simulink model "MATLAB_TEST"  (R2019b)
settings: Solver=FixedStepDiscrete  StartTime=0  StopTime=50  FixedStep=0.0025  RelTol=1e-3
undefined symbols (not defined in the file): BCM_COM_PROC_P20, BCM_COM_PROC_P20_SFW_R2018b, BCM_COM_PROC_P2_5, BCM_COM_PROC_P2_5_SFW_R2018b, BCM_COM_PROC_P5, BCM_COM_PROC_P5_SFW_R2018b, BCMA_ACCU_PT_Conf_Flt, BCMA_ACCU_PT_Unconf_Flt, BCMA_Antiskid_Off_Sanction, BCMA_Avionics_Conf_Flt, BCMA_BCM_CCDL_Conf_Flt, BCMA_BCM_CCDL_Unconf_Flt, BCMA_BCM_DBCU_INHIBITION_Conf_Flt, BCMA_BCM_DBCU_INHIBITION_Unconf_Flt, BCMA_BCP_ALT_Disp_Sw_Conf_Flt, BCMA_BCP_ALT_Disp_Sw_Unconf_Flt, BCMA_BCP_ALT_SW_ON_CMD_Conf_Flt, BCMA_BCP_ALT_SW_ON_CMD_Unconf_Flt, BCMA_BCP_PARK_OFF_SW_CMD_Conf_Flt, BCMA_BCP_PARK_OFF_SW_CMD_Unconf_Flt, BCMA_CF_BSELV_JCL, BCMA_CF_BSELV_JOP, BCMA_CF_BSELV_OC, BCMA_CF_BSELV_SC, BCMA_CF_LH_SV_JCL, BCMA_CF_LH_SV_JOP, BCMA_CF_LH_SV_OC, BCMA_CF_LH_SV_SC, BCMA_CF_PARK_BRK, BCMA_CF_RESIDUAL_PRESS, BCMA_CF_RH_SV_JCL, BCMA_CF_RH_SV_JOP, BCMA_CF_RH_SV_OC, BCMA_CF_RH_SV_SC, BCMA_CF_SELV_JCL, BCMA_CF_SELV_JOP, BCMA_CF_SELV_OC, BCMA_CF_SELV_SC, BCMA_CF_SV_DRIFT, BCMA_DBCU_ALT_MODE_Conf_Flt, BCMA_DBCU_ALT_MODE_Unconf_Flt, BCMA_DBCU_BRK_ORDER_FAIL_Conf_Flt, BCMA_DBCU_BRK_ORDER_FAIL_Unconf_Flt, BCMA_DBCU_Conf_Flt, BCMA_DBCU_DISPATCH_SW_ON_Conf_Flt, BCMA_DBCU_DISPATCH_SW_ON_Unconf_Flt, BCMA_DBCU_FAILED_Conf_Flt, BCMA_DBCU_FAILED_Unconf_Flt, BCMA_DFCS1_Capsule_Validity, BCMA_DFCS1_Label202_Corrupted, BCMA_DFCS1_Label202_Not_Refreshed, BCMA_DFCS1_Label204_Corrupted, BCMA_DFCS1_Label204_Not_Refreshed, BCMA_DFCS1_Label205_Corrupted, BCMA_DFCS1_Label205_Not_Refreshed, BCMA_DFCS1_Label206_Corrupted, BCMA_DFCS1_Label206_Not_Refreshed, BCMA_DFCS1_Label207_Corrupted, BCMA_DFCS1_Label207_Not_Refreshed, BCMA_DFCS3_Capsule_Validity ... (+762)
libraries: simulink x73, lib_MBD_Control x5
(part 5 of 16)

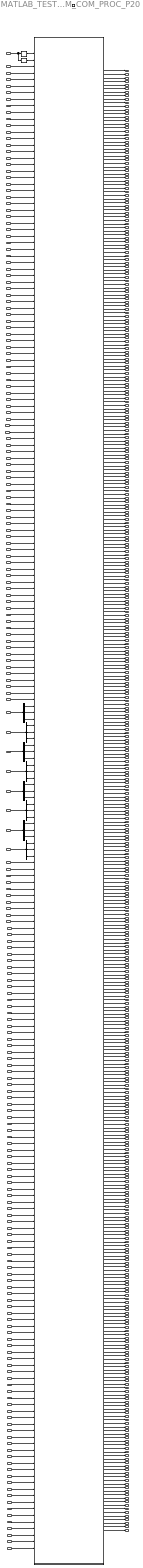
== system MATLAB_TEST/AVIONICS/Brake_Control_Module_Side_A/BCSA Controller CP/BCM_COM_PROC_P20 ==
  V_BCM_COM_Tachometers_Conf_Flt : Inport
  V_BCM_COM_DFCS_A_Gnd_Spd_Acq : Inport  Port=2
  V_BCM_COM_DFCS_B_Gnd_Spd_Acq : Inport  Port=3
  V_BCM_COM_DFCS_A_Gnd_Spd_Val : Inport  Port=4
  V_BCM_COM_DFCS_B_Gnd_Spd_Val : Inport  Port=5
  V_BCM_COM_DFCS_A_Long_Accel_Acq : Inport  Port=6
  V_BCM_COM_DFCS_B_Long_Accel_Acq : Inport  Port=7
  V_BCM_COM_DFCS_A_AC_Long_Accel_Val : Inport  Port=8
  V_BCM_COM_DFCS_B_AC_Long_Accel_Val : Inport  Port=9
  V_BCM_COM_DFCS_A_Pitch_Ang_Acq : Inport  Port=10
  V_BCM_COM_DFCS_B_Pitch_Ang_Acq : Inport  Port=11
  V_BCM_COM_DFCS_A_AC_Pitch_Angle_Val : Inport  Port=12
  V_BCM_COM_DFCS_B_AC_Pitch_Angle_Val : Inport  Port=13
  V_BCM_COM_DFCS_A_WOWs_Val_Acq : Inport  Port=14
  V_BCM_COM_DFCS_B_WOWs_Val_Acq : Inport  Port=15
  V_BCM_COM_DFCS_A_WOWs_Val_Val : Inport  Port=16
  V_BCM_COM_DFCS_B_WOWs_Val_Val : Inport  Port=17
  V_BCM_COM_DFCS_A_LMLG_WOWs_Val : Inport  Port=18
  V_BCM_COM_DFCS_B_LMLG_WOWs_Val : Inport  Port=19
  V_BCM_COM_DFCS_A_LMLG_WOWs_Acq : Inport  Port=20
  V_BCM_COM_DFCS_B_LMLG_WOWs_Acq : Inport  Port=21
  V_BCM_COM_DFCS_A_RMLG_WOWs_Val : Inport  Port=22
  V_BCM_COM_DFCS_B_RMLG_WOWs_Val : Inport  Port=23
  V_BCM_COM_DFCS_A_RMLG_WOWs_Acq : Inport  Port=24
  V_BCM_COM_DFCS_B_RMLG_WOWs_Acq : Inport  Port=25
  V_BCM_COM_DFCS_A_NLG_WOWs_Val : Inport  Port=26
  V_BCM_COM_DFCS_B_NLG_WOWs_Val : Inport  Port=27
  V_BCM_COM_DFCS_A_NLG_WOWs_Acq : Inport  Port=28
  V_BCM_COM_DFCS_B_NLG_WOWs_Acq : Inport  Port=29
  V_BCM_COM_RH_Decel_Law_Brkg_Press_Cmd : Inport  Port=30
  V_BCM_COM_LH_Decel_Law_Brkg_Press_Cmd : Inport  Port=31
  V_BCM_COM_Hyd_A_Press_Acq : Inport  Port=32
  V_BCM_COM_Hyd_B_Press_Acq : Inport  Port=33
  V_BCM_COM_DFCS_A_LH_Braking_Cmd_Val : Inport  Port=34
  V_BCM_COM_DFCS_A_RH_Braking_Cmd_Val : Inport  Port=35
  V_BCM_COM_DFCS_B_LH_Braking_Cmd_Val : Inport  Port=36
  V_BCM_COM_DFCS_B_RH_Braking_Cmd_Val : Inport  Port=37
  V_BCM_COM_DFCS_A_DFCS_LH_Braking_Cmd_Acq : Inport  Port=38
  V_BCM_COM_DFCS_A_DFCS_RH_Braking_Cmd_Acq : Inport  Port=39
  V_BCM_COM_DFCS_B_DFCS_LH_Braking_Cmd_Acq : Inport  Port=40
  V_BCM_COM_DFCS_B_DFCS_RH_Braking_Cmd_Acq : Inport  Port=41
  V_BCM_COM_DFCS_A_Decel_Law_Inhib_Val : Inport  Port=42
  V_BCM_COM_DFCS_A_Decel_Law_Inhib_Acq : Inport  Port=43
  V_BCM_COM_DFCS_B_Decel_Law_Inhib_Val : Inport  Port=44
  V_BCM_COM_DFCS_B_Decel_Law_Inhib_Acq : Inport  Port=45
  V_BCM_COM_DFCS_A_TLA_Above_Idle_Val : Inport  Port=46
  V_BCM_COM_DFCS_B_TLA_Above_Idle_Val : Inport  Port=47
  V_BCM_COM_DFCS_A_TLA_Above_Idle_Acq : Inport  Port=48
  V_BCM_COM_DFCS_B_TLA_Above_Idle_Acq : Inport  Port=49
  V_BCM_COM_LG_Lever_Up_Acq : Inport  Port=50
  V_BCM_COM_LG_Lever_Up_Unconf_Flt : Inport  Port=51
  V_BCM_COM_LG_Lever_Up_Conf_Flt : Inport  Port=52
  V_BCM_COM_LMLG_Downlock_Acq : Inport  Port=53
  V_BCM_COM_RMLG_Downlock_Acq : Inport  Port=54
  V_BCM_COM_LMLG_Dnlk_Unconf_Flt : Inport  Port=55
  V_BCM_COM_LMLG_Dnlk_Conf_Flt : Inport  Port=56
  V_BCM_COM_RMLG_Dnlk_Unconf_Flt : Inport  Port=57
  V_BCM_COM_RMLG_Dnlk_Conf_Flt : Inport  Port=58
  V_BCM_COM_Engine_Running_Acq : Inport  Port=59
  V_BCM_COM_PBSELV_ON_POS_Acq : Inport  Port=60
  V_BCM_COM_PBSELV_ON_POS_Unconf_Flt : Inport  Port=61
  V_BCM_COM_PBSELV_ON_POS_Conf_Flt : Inport  Port=62
  V_BCM_COM_Maint_Itv_Function_Req : Inport  Port=63
  V_BCM_COM_BCM_Config : Inport  Port=64
  V_BCM_COM_BCM_Off_Sanction : Inport  Port=65
  V_BCM_COM_BCM_Validity_By_SP : Inport  Port=66
  V_BCM_COM_BCP_BCM_Alt_Sw_On_Cmd_Acq : Inport  Port=67
  V_BCM_COM_BCP_BCM_Alt_Sw_On_Cmd_Conf_Flt : Inport  Port=68
  V_BCM_COM_BCP_BCM_Alt_Sw_On_Cmd_Unconf_Flt : Inport  Port=69
  V_BCM_COM_MP_BCMA_Alt_Disp_Sw_Conf_Flt : Inport  Port=70
  V_BCM_COM_MP_BCMA_Alt_Disp_Sw_Unconf_Flt : Inport  Port=71
  V_BCM_COM_MP_BCMA_Alt_Disp_Sw_Acq : Inport  Port=72
  V_BCM_COM_Antiskid_Off_Sanction : Inport  Port=73
  V_BCM_COM_Norm_Brkg_Off_Sanc : Inport  Port=74
  V_BCM_COM_CF_LH_ALT_BRK_LOSS : Inport  Port=75
  V_BCM_COM_CF_DBCU_FAILED : Inport  Port=76
  V_BCM_COM_CF_RH_ALT_BRK_LOSS : Inport  Port=77
  V_BCM_COM_SV_PT_Filt : Inport  Port=78
  V_BCM_COM_Whl_AS_Inhib_Cond_W12 : Inport  Port=79
  V_BCM_COM_Whl_AS_Inhib_Cond_W34 : Inport  Port=80
  V_BCM_COM_Whl_LP_AS_Curr_Order : Inport  Port=81
  V_BCM_COM_SV_PT_Cons : Inport  Port=82
  V_BCM_COM_Wheel_Filtered_Speed_W12 : Inport  Port=83
  V_BCM_COM_Wheel_Filtered_Speed_W34 : Inport  Port=84
  V_BCM_COM_Wheel_Speed_Error_W12 : Inport  Port=85
  V_BCM_COM_Wheel_Speed_Error_W34 : Inport  Port=86
  V_BCM_COM_Whl_LP_AS_Curr_Order_W12 : Inport  Port=87
  V_BCM_COM_Whl_LP_AS_Curr_Order_W34 : Inport  Port=88
  V_BCM_COM_SV_Current : Inport  Port=89
  V_BCM_COM_SV_PT_Cons_Val : Inport  Port=90
  V_BCM_COM_Opt_Adhesion_In_Acq_W12 : Inport  Port=91
  V_BCM_COM_Opt_Adhesion_In_Acq_W34 : Inport  Port=92
  V_BCM_COM_Adhesion_In_Acq_W12 : Inport  Port=93
  V_BCM_COM_Adhesion_In_Acq_W34 : Inport  Port=94
  V_BCM_COM_Target_Speed_In_Acq_W12 : Inport  Port=95
  V_BCM_COM_Target_Speed_In_Acq_W34 : Inport  Port=96
  V_BCM_COM_Big_Gamma_Trig_In_Acq_W12 : Inport  Port=97
  V_BCM_COM_Big_Gamma_Trig_In_Acq_W34 : Inport  Port=98
  V_BCM_COM_Small_Slip_Trig_In_Acq_W12 : Inport  Port=99
  V_BCM_COM_Small_Slip_Trig_In_Acq_W34 : Inport  Port=100
  V_BCM_COM_Big_Slip_Trig_In_Acq_W12 : Inport  Port=101
  V_BCM_COM_Big_Slip_Trig_In_Acq_W34 : Inport  Port=102
  V_BCM_COM_BCM_CCDL_Conf_Flt : Inport  Port=103
  V_BCM_COM_BCM_CCDL_Unconf_Flt : Inport  Port=104
  V_BCM_COM_Big_Slip_WD_Trig_In_Acq_W12 : Inport  Port=105
  V_BCM_COM_Big_Slip_WD_Trig_In_Acq_W34 : Inport  Port=106
  V_BCM_COM_BCM_DBCU_INHIBITION_Conf_Flt : Inport  Port=107
  V_BCM_COM_BCM_DBCU_INHIBITION_Unconf_Flt : Inport  Port=108
  V_BCM_COM_BCM_DBCU_INHIBITION_Acq : Inport  Port=109
  V_BCM_COM_Engine_1_Running_Acq_Val : Inport  Port=110
  V_BCM_COM_Engine_2_Running_Acq_Val : Inport  Port=111
  V_BCM_COM_Hyd_A_Press_Acq_Val : Inport  Port=112
  V_BCM_COM_Hyd_B_Press_Acq_Val : Inport  Port=113
  V_BCM_COM_DFCS_A_DBCU_ALT_Mode_1_Acq_Val : Inport  Port=114
  V_BCM_COM_DFCS_A_DBCU_ALT_Mode_2_Acq_Val : Inport  Port=115
  V_BCM_COM_DFCS_B_DBCU_ALT_Mode_1_Acq_Val : Inport  Port=116
  V_BCM_COM_DFCS_B_DBCU_ALT_Mode_2_Acq_Val : Inport  Port=117
  V_BCM_COM_UTC_Time_Hours_Acq : Inport  Port=118
  V_BCM_COM_UTC_Time_Hours_Conf_Flt : Inport  Port=119
  V_BCM_COM_UTC_Time_Hours_Unconf_Flt : Inport  Port=120
  V_BCM_COM_UTC_Time_Minutes_Acq : Inport  Port=121
  V_BCM_COM_UTC_Time_Minutes_Conf_Flt : Inport  Port=122
  V_BCM_COM_UTC_Time_Minutes_Unconf_Flt : Inport  Port=123
  V_BCM_COM_UTC_Time_Seconds_Acq : Inport  Port=124
  V_BCM_COM_UTC_Time_Seconds_Conf_Flt : Inport  Port=125
  V_BCM_COM_UTC_Time_Seconds_Unconf_Flt : Inport  Port=126
  V_BCM_COM_DBCU_BRK_ORDER_FAIL_Acq : Inport  Port=127
  V_BCM_COM_DBCU_DISPATCH_SW_ON_Acq : Inport  Port=128
  V_BCM_COM_LH_DBCU_BRK_CMD_FDBK_Acq : Inport  Port=129
  V_BCM_COM_RH_DBCU_BRK_CMD_FDBK_Acq : Inport  Port=130
  V_BCM_COM_DBCU_FAILED_Acq : Inport  Port=131
  V_BCM_COM_DBCU_ALT_MODE_Acq : Inport  Port=132
  V_BCM_COM_DBCU_BRK_ORDER_FAIL_Conf_Flt : Inport  Port=133
  V_BCM_COM_DBCU_BRK_ORDER_FAIL_Unconf_Flt : Inport  Port=134
  V_BCM_COM_DBCU_DISPATCH_SW_ON_Conf_Flt : Inport  Port=135
  V_BCM_COM_DBCU_DISPATCH_SW_ON_Unconf_Flt : Inport  Port=136
  V_BCM_COM_LH_DBCU_BRK_CMD_FDBK_Conf_Flt : Inport  Port=137
  V_BCM_COM_LH_DBCU_BRK_CMD_FDBK_Unconf_Flt : Inport  Port=138
  V_BCM_COM_RH_DBCU_BRK_CMD_FDBK_Conf_Flt : Inport  Port=139
  V_BCM_COM_RH_DBCU_BRK_CMD_FDBK_Unconf_Flt : Inport  Port=140
  V_BCM_COM_DBCU_FAILED_Conf_Flt : Inport  Port=141
  V_BCM_COM_DBCU_FAILED_Unconf_Flt : Inport  Port=142
  V_BCM_COM_DBCU_ALT_MODE_Conf_Flt : Inport  Port=143
  V_BCM_COM_DBCU_ALT_MODE_Unconf_Flt : Inport  Port=144
  V_BCM_COM_ACCU_PT_Conf_Flt : Inport  Port=145
  V_BCM_COM_ACCU_PT_Unconf_Flt : Inport  Port=146
  V_BCM_COM_ACCU_PT_Acq : Inport  Port=147
  V_BCM_COM_LH_BTS_TEMP_Comp : Inport  Port=148
  V_BCM_COM_LH_BTS_Conf_Flt : Inport  Port=149
  V_BCM_COM_LH_BTS_Unconf_Flt : Inport  Port=150
  V_BCM_COM_RH_BTS_TEMP_Comp : Inport  Port=151
  V_BCM_COM_RH_BTS_Conf_Flt : Inport  Port=152
  V_BCM_COM_RH_BTS_Unconf_Flt : Inport  Port=153
  V_BCM_COM_BCP_PARK_OFF_SW_CMD_Acq : Inport  Port=154
  V_BCM_COM_BCP_PARK_OFF_SW_CMD_Conf_Flt : Inport  Port=155
  V_BCM_COM_BCP_PARK_OFF_SW_CMD_Unconf_Flt : Inport  Port=156
  V_BCM_COM_MP_MAINT_MODE_CMD_28V_Acq : Inport  Port=157
  V_BCM_COM_MP_MAINT_MODE_CMD_GND_Acq : Inport  Port=158
  V_BCM_COM_LNLG_Tire_Press_Acq : Inport  Port=159
  V_BCM_COM_LNLG_Tire_Press_Conf_Flt : Inport  Port=160
  V_BCM_COM_LNLG_Tire_Press_Unconf_Flt : Inport  Port=161
  V_BCM_COM_RNLG_Tire_Press_Acq : Inport  Port=162
  V_BCM_COM_RNLG_Tire_Press_Conf_Flt : Inport  Port=163
  V_BCM_COM_RNLG_Tire_Press_Unconf_Flt : Inport  Port=164
  V_BCM_COM_LMLG_Outboard_Tire_Press_Acq : Inport  Port=165
  V_BCM_COM_LMLG_Outboard_Tire_Press_Conf_Flt : Inport  Port=166
  V_BCM_COM_LMLG_Outboard_Tire_Press_Unconf_Flt : Inport  Port=167
  V_BCM_COM_LMLG_Inboard_Tire_Press_Acq : Inport  Port=168
  V_BCM_COM_LMLG_Inboard_Tire_Press_Conf_Flt : Inport  Port=169
  V_BCM_COM_LMLG_Inboard_Tire_Press_Unconf_Flt : Inport  Port=170
  V_BCM_COM_RMLG_Inboard_Tire_Press_Acq : Inport  Port=171
  V_BCM_COM_RMLG_Inboard_Tire_Press_Conf_Flt : Inport  Port=172
  V_BCM_COM_RMLG_Inboard_Tire_Press_Unconf_Flt : Inport  Port=173
  V_BCM_COM_RMLG_Outboard_Tire_Press_Acq : Inport  Port=174
  V_BCM_COM_RMLG_Outboard_Tire_Press_Conf_Flt : Inport  Port=175
  V_BCM_COM_RMLG_Outboard_Tire_Press_Unconf_Flt : Inport  Port=176
  V_BCM_COM_Whl_AS_Curr_Order : Inport  Port=177
  V_BCM_COM_SV_Current_Readback : Inport  Port=178
  V_BCM_COM_Whl_AS_Activity : Inport  Port=179
  V_BCM_COM_SELV_High_Side_Readback_Val : Inport  Port=180
  V_BCM_COM_SELV_High_Side_Readback : Inport  Port=181
  V_BCM_COM_CF_LH_SV_SC : Inport  Port=182
  V_BCM_COM_CF_LH_SV_OC : Inport  Port=183
  V_BCM_COM_CF_RH_SV_SC : Inport  Port=184
  V_BCM_COM_CF_RH_SV_OC : Inport  Port=185
  V_BCM_COM_CF_SELV_SC : Inport  Port=186
  V_BCM_COM_CF_SELV_OC : Inport  Port=187
  V_BCM_COM_CF_SELV_JOP : Inport  Port=188
  V_BCM_COM_CF_SELV_JCL : Inport  Port=189
  V_BCM_COM_CF_PARK_BRK : Inport  Port=190
  V_BCM_COM_CF_RESIDUAL_PRESS : Inport  Port=191
  V_BCM_COM_Avionics_Conf_Flt : Inport  Port=192
  V_BCM_COM_DFCS_A_Conf_Flt : Inport  Port=193
  V_BCM_COM_DFCS_A_DFCS_BCM_Caps_Val : Inport  Port=194
  V_BCM_COM_DFCS_B_Conf_Flt : Inport  Port=195
  V_BCM_COM_DFCS_B_DFCS_BCM_Caps_Val : Inport  Port=196
  V_BCM_COM_PPRG_i_Acquired : Inport  Port=197
  V_BCM_COM_PPRG_Fault : Inport  Port=198
  V_BCM_COM_DBCU_Conf_Flt : Inport  Port=199
  V_BCM_COM_SV_Current_Readback_Val : Inport  Port=200
  V_BCM_COM_SV_Current_Order : Inport  Port=201
  V_BCM_COM_CF_BSELV_OC : Inport  Port=202
  V_BCM_COM_CF_BSELV_SC : Inport  Port=203
  V_BCM_COM_CF_BSELV_JCL : Inport  Port=204
  V_BCM_COM_CF_BSELV_JOP : Inport  Port=205
  V_BCM_COM_LH_SV_PT_Conf_Flt : Inport  Port=206
  V_BCM_COM_CF_SV_DRIFT : Inport  Port=207
  V_BCM_COM_CF_LH_SV_JCL : Inport  Port=208
  V_BCM_COM_CF_LH_SV_JOP : Inport  Port=209
  V_BCM_COM_RH_SV_PT_Conf_Flt : Inport  Port=210
  V_BCM_COM_CF_RH_SV_JCL : Inport  Port=211
  V_BCM_COM_CF_RH_SV_JOP : Inport  Port=212
  BCM_Tuning : Inport  Port=213
  Enable : EnablePort  StatesWhenEnabling=reset
      settings: AttributesFormatString=StatesWhenEnabling %<StatesWhenEnabling>
  BCM_COM_PROC_P20 : Subsystem  Priority=3  AncestorBlock=BCM_COM_PROC_P20_SFW_R2018b/BCM_COM_PROC_P20  TreatAsAtomicUnit=on  SystemSampleTime=0.02
  Demux{,1..7} (8 alike) : Demux  Outputs=3
  Selector : Selector  InputPortWidth=4  IndexOptions=Index vector (dialog)  Indices=[1 2]  OutputSizes=1
  Selector1 : Selector  InputPortWidth=4  IndexOptions=Index vector (dialog)  Indices=[3 4]  OutputSizes=1
  V_BCM_COM_Whl_Spun_Up_State_W12 : Outport
  V_BCM_COM_Whl_Ref_Speed_W12 : Outport  Port=2
  V_BCM_COM_Whl_Spun_Up_State_W34 : Outport  Port=3
  V_BCM_COM_Whl_Ref_Speed_W34 : Outport  Port=4
  V_BCM_COM_DFCS_A_Gnd_Spd_Conv : Outport  Port=5
  V_BCM_COM_DFCS_B_Gnd_Spd_Conv : Outport  Port=6
  V_BCM_COM_AC_Gnd_Spd_Cons : Outport  Port=7
  V_BCM_COM_AC_Gnd_Spd_Cons_Val : Outport  Port=8
  V_BCM_COM_DFCS_A_Long_Accel_Conv : Outport  Port=9
  V_BCM_COM_DFCS_B_Long_Accel_Conv : Outport  Port=10
  V_BCM_COM_AC_Long_Accel_Cons : Outport  Port=11
  V_BCM_COM_AC_Long_Accel_Cons_Val : Outport  Port=12
  V_BCM_COM_AC_Long_Accel_Filt_Corr : Outport  Port=13
  V_BCM_COM_AC_Pitch_Ang_Cons_Val : Outport  Port=14
  V_BCM_COM_AC_Pitch_Ang_Filt : Outport  Port=15
  V_BCM_COM_AC_Pitch_Ang_Cons : Outport  Port=16
  V_BCM_COM_DFCS_A_WOWs_Val_Cons : Outport  Port=17
  V_BCM_COM_DFCS_B_WOWs_Val_Cons : Outport  Port=18
  V_BCM_COM_LMLG_WOWs_Cons : Outport  Port=19
  V_BCM_COM_LMLG_WOWs_Cons_Val : Outport  Port=20
  V_BCM_COM_RMLG_WOWs_Cons : Outport  Port=21
  V_BCM_COM_RMLG_WOWs_Cons_Val : Outport  Port=22
  V_BCM_COM_NLG_WOWs_Cons : Outport  Port=23
  V_BCM_COM_NLG_WOWs_Cons_Val : Outport  Port=24
  V_BCM_COM_LMLG_On_Gnd_State : Outport  Port=25
  V_BCM_COM_RMLG_On_Gnd_State : Outport  Port=26
  V_BCM_COM_LMLG_On_Gnd_State_Val : Outport  Port=27
  V_BCM_COM_RMLG_On_Gnd_State_Val : Outport  Port=28
  V_BCM_COM_MLG_On_Gnd_State : Outport  Port=29
  V_BCM_COM_NLG_On_Gnd_State : Outport  Port=30
  V_BCM_COM_NLG_On_Gnd_State_Val : Outport  Port=31
  V_BCM_COM_NLG_On_Gnd_State_Cons : Outport  Port=32
  V_BCM_COM_LH_Braking_Cmd_Cons : Outport  Port=33
  V_BCM_COM_RH_Braking_Cmd_Cons : Outport  Port=34
  V_BCM_COM_Decel_Law_Inhib_Cons : Outport  Port=35
  V_BCM_COM_Decel_Law_Inhib_Cons_Val : Outport  Port=36
  V_BCM_COM_TLA_State_Cons : Outport  Port=37
  V_BCM_COM_TLA_State_Cons_Val : Outport  Port=38
  V_BCM_COM_LG_Lever_Up_Conf : Outport  Port=39
  V_BCM_COM_LG_Lever_State_Cons : Outport  Port=40
  V_BCM_COM_LG_Lever_Ste_Cons_Val : Outport  Port=41
  V_BCM_COM_LMLG_Downlock_Conf : Outport  Port=42
  V_BCM_COM_RMLG_Downlock_Conf : Outport  Port=43
  V_BCM_COM_LMLG_Downlock_State : Outport  Port=44
  V_BCM_COM_LMLG_Dnlk_State_Val : Outport  Port=45
  V_BCM_COM_RMLG_Downlock_State : Outport  Port=46
  V_BCM_COM_RMLG_Dnlk_State_Val : Outport  Port=47
  V_BCM_COM_SELV_High_Side_Cmd_Order : Outport  Port=48
  V_BCM_COM_SELV_Low_Speed_Logic : Outport  Port=49
  V_BCM_COM_Engine_State : Outport  Port=50
  V_BCM_COM_Engine_State_Val : Outport  Port=51
  V_BCM_COM_LH_Braking_Cmd_State : Outport  Port=52
  V_BCM_COM_RH_Braking_Cmd_State : Outport  Port=53
  V_BCM_COM_LH_Regular_Brkg_Press_Cmd : Outport  Port=54
  V_BCM_COM_RH_Regular_Brkg_Press_Cmd : Outport  Port=55
  V_BCM_COM_Wheels_Global_Spun_Up_Ste : Outport  Port=56
  V_BCM_COM_Global_Reference_Spd : Outport  Port=57
  V_BCM_COM_Global_Wheel_Spd : Outport  Port=58
  V_BCM_COM_LMLG_Global_Wheel_Spd : Outport  Port=59
  V_BCM_COM_RMLG_Global_Wheel_Spd : Outport  Port=60
  V_BCM_COM_AC_State : Outport  Port=61
  V_BCM_COM_AC_Flight_Phase : Outport  Port=62
  V_BCM_COM_Braking_Mode : Outport  Port=63
  v_BCM_COM_FT_Seq : Outport  Port=64
  V_BCM_COM_Start_Norm_FT_Cond : Outport  Port=65
  V_BCM_COM_Brkg_Norm_FT_Prog_Sts : Outport  Port=66
  V_BCM_COM_Brkg_Norm_FT_Cond : Outport  Port=67
  V_BCM_COM_Braking_Norm_FT_Seq : Outport  Port=68
  V_BCM_COM_Abort_Norm_FT_Cond : Outport  Port=69
  V_BCM_COM_Brkg_Alt_FT_Prog_Sts : Outport  Port=70
  V_BCM_COM_Braking_Alt_FT_Seq : Outport  Port=71
  V_BCM_COM_Abort_Alt_FT_Cond : Outport  Port=72
  V_BCM_COM_Start_Alt_FT_Cond : Outport  Port=73
  V_BCM_COM_Brkg_Alt_FT_Cond : Outport  Port=74
  V_BCM_COM_LH_Press_Reg_FT_Act_Cond : Outport  Port=75
  V_BCM_COM_RH_Press_Reg_FT_Act_Cond : Outport  Port=76
  V_BCM_COM_LH_Press_Law_Brkg_Press_Cmd : Outport  Port=77
  V_BCM_COM_RH_Press_Law_Brkg_Press_Cmd : Outport  Port=78
  V_BCM_COM_LH_FT_Press_Cmd : Outport  Port=79
  V_BCM_COM_RH_FT_Press_Cmd : Outport  Port=80
  V_BCM_COM_LH_Ret_Brkg_Press_Cmd : Outport  Port=81
  V_BCM_COM_RH_Ret_Brkg_Press_Cmd : Outport  Port=82
  V_BCM_COM_LH_Eng_Run_Press_Cmd : Outport  Port=83
  V_BCM_COM_RH_Eng_Run_Press_Cmd : Outport  Port=84
  V_BCM_COM_Brkg_SELV_High_Side_FT_Cmd_Order : Outport  Port=85
  V_BCM_COM_DBCU_FT_Inhib_Order : Outport  Port=86
  V_BCM_COM_DBCU_Inhib_Order : Outport  Port=87
  V_BCM_COM_BCM_Validity : Outport  Port=88
  V_BCM_COM_Alt_Sw_Cmd_Cons : Outport  Port=89
  V_BCM_COM_Alt_Sw_Cmd_Cons_Val : Outport  Port=90
  V_BCM_COM_Disp_Sw_Cmd_Cons : Outport  Port=91
  V_BCM_COM_Disp_Sw_Cmd_Cons_Val : Outport  Port=92
  V_BCM_COM_MP_BCMA_Alt_Disp_Sw_Conf : Outport  Port=93
  V_BCM_COM_BCP_BCM_Alt_Sw_On_Cmd_Conf : Outport  Port=94
  V_BCM_COM_Braking_State : Outport  Port=95
  V_BCM_COM_Norm_Brkg_Availability : Outport  Port=96
  V_BCM_COM_Alt_Brkg_Availability : Outport  Port=97
  V_BCM_COM_Braking_Type : Outport  Port=98
  V_BCM_COM_Press_Cmd : Outport  Port=99
  V_BCM_COM_Brkg_On_Wheels : Outport  Port=100
  V_BCM_COM_Press_Cmd_Rate_Lim : Outport  Port=101
  V_BCM_COM_PBSELV_ON_POS_Conf : Outport  Port=102
  V_BCM_COM_PBSELV_State_Cons : Outport  Port=103
  V_BCM_COM_PBSELV_State_Cons_Val : Outport  Port=104
  V_BCM_COM_Hyd_A_Press_Cons : Outport  Port=105
  V_BCM_COM_Hyd_B_Press_Cons : Outport  Port=106
  V_BCM_COM_Hyd_A_Press_Cons_Val : Outport  Port=107
  V_BCM_COM_Hyd_B_Press_Cons_Val : Outport  Port=108
  V_BCM_COM_Hyd_A_Press_State : Outport  Port=109
  V_BCM_COM_Hyd_B_Press_State : Outport  Port=110
  V_BCM_COM_Sys_Sanc_Inhib_During_FT : Outport  Port=111
  V_BCM_COM_Wheel_Control_Speed_W12 : Outport  Port=112
  V_BCM_COM_Wheel_Control_Speed_W34 : Outport  Port=113
  V_BCM_COM_Big_Gamma_Trig_Out_W12 : Outport  Port=114
  V_BCM_COM_Big_Gamma_Trig_Out_W34 : Outport  Port=115
  V_BCM_COM_Big_Slip_Trig_Out_W12 : Outport  Port=116
  V_BCM_COM_Big_Slip_Trig_Out_W34 : Outport  Port=117
  V_BCM_COM_Big_Slip_WD_Trig_Out_W12 : Outport  Port=118
  V_BCM_COM_Big_Slip_WD_Trig_Out_W34 : Outport  Port=119
  V_BCM_COM_Small_Slip_Trig_Out_W12 : Outport  Port=120
  V_BCM_COM_Small_Slip_Trig_Out_W34 : Outport  Port=121
  V_BCM_COM_Automate_State_W12 : Outport  Port=122
  V_BCM_COM_Automate_State_W34 : Outport  Port=123
  V_BCM_COM_Target_Speed_Out_W12 : Outport  Port=124
  V_BCM_COM_Target_Speed_Out_W34 : Outport  Port=125
  V_BCM_COM_Target_Decel_Out_W12 : Outport  Port=126
  V_BCM_COM_Target_Decel_Out_W34 : Outport  Port=127
  V_BCM_COM_Adhesion_Out_W12 : Outport  Port=128
  V_BCM_COM_Adhesion_Out_W34 : Outport  Port=129
  V_BCM_COM_Opt_Adhesion_Out_W12 : Outport  Port=130
  V_BCM_COM_Opt_Adhesion_Out_W34 : Outport  Port=131
  V_BCM_COM_Whl_AS_Adp_Gain_W12 : Outport  Port=132
  V_BCM_COM_Whl_AS_Adp_Gain_W34 : Outport  Port=133
  V_BCM_COM_Adhesion_In_Cons_W12 : Outport  Port=134
  V_BCM_COM_Adhesion_In_Cons_W34 : Outport  Port=135
  V_BCM_COM_Opt_Adhesion_In_Cons_W12 : Outport  Port=136
  V_BCM_COM_Opt_Adhesion_In_Cons_W34 : Outport  Port=137
  V_BCM_COM_Target_Speed_In_Cons_W12 : Outport  Port=138
  V_BCM_COM_Target_Speed_In_Cons_W34 : Outport  Port=139
  V_BCM_COM_Big_Slip_WD_Trig_In_Cons_W12 : Outport  Port=140
  V_BCM_COM_Big_Slip_WD_Trig_In_Cons_W34 : Outport  Port=141
  V_BCM_COM_Big_Gamma_Trig_In_Cons_W12 : Outport  Port=142
  V_BCM_COM_Big_Gamma_Trig_In_Cons_W34 : Outport  Port=143
  V_BCM_COM_Small_Slip_Trig_In_Cons_W12 : Outport  Port=144
  V_BCM_COM_Small_Slip_Trig_In_Cons_W34 : Outport  Port=145
  V_BCM_COM_Big_Slip_Trig_In_Cons_W12 : Outport  Port=146
  V_BCM_COM_Big_Slip_Trig_In_Cons_W34 : Outport  Port=147
  V_BCM_COM_CCDL_Data_From_Opp_BCM_Val : Outport  Port=148
  V_BCM_COM_DBCU_Inhibition_Order_From_Opp_BCM_Cons : Outport  Port=149
  V_BCM_COM_DBCU_Inhibition_Order_From_Opp_BCM_Cons_Val : Outport  Port=150
  V_BCM_COM_Engine_Running_Conf_Flt : Outport  Port=151
  V_BCM_COM_Engine_Running_Unconf_Flt : Outport  Port=152
  V_BCM_COM_Hyd_A_Press_Conf_Flt : Outport  Port=153
  V_BCM_COM_Hyd_B_Press_Conf_Flt : Outport  Port=154
  V_BCM_COM_Hyd_A_Press_Unconf_Flt : Outport  Port=155
  V_BCM_COM_Hyd_B_Press_Unconf_Flt : Outport  Port=156
  V_BCM_COM_DFCS_A_AC_Gnd_Spd_Val : Outport  Port=157
  V_BCM_COM_DFCS_A_AC_Long_Accel_Val1 : Outport  Port=158
  V_BCM_COM_DFCS_A_AC_Pitch_Angle_Val1 : Outport  Port=159
  V_BCM_COM_DFCS_A_Decel_Law_Inhib_Val1 : Outport  Port=160
  V_BCM_COM_DFCS_B_Decel_Law_Inhib_Val1 : Outport  Port=161
  V_BCM_COM_DFCS_B_AC_Gnd_Spd_Val : Outport  Port=162
  V_BCM_COM_DFCS_B_AC_Long_Accel_Val1 : Outport  Port=163
  V_BCM_COM_DFCS_B_AC_Pitch_Angle_Val1 : Outport  Port=164
  V_BCM_COM_DFCS_A_LMLG_WOWs_Val1 : Outport  Port=165
  V_BCM_COM_DFCS_A_RMLG_WOWs_Val1 : Outport  Port=166
  V_BCM_COM_DFCS_A_NLG_WOWs_Val1 : Outport  Port=167
  V_BCM_COM_DFCS_A_WOWs_Val_Val1 : Outport  Port=168
  V_BCM_COM_DFCS_B_LMLG_WOWs_Val1 : Outport  Port=169
  V_BCM_COM_DFCS_B_RMLG_WOWs_Val1 : Outport  Port=170
  V_BCM_COM_DFCS_B_NLG_WOWs_Val1 : Outport  Port=171
  V_BCM_COM_DFCS_B_WOWs_Val_Val1 : Outport  Port=172
  V_BCM_COM_DFCS_A_LH_Braking_Cmd_Val1 : Outport  Port=173
  V_BCM_COM_DFCS_A_RH_Braking_Cmd_Val1 : Outport  Port=174
  V_BCM_COM_DFCS_B_LH_Braking_Cmd_Val1 : Outport  Port=175
  V_BCM_COM_DFCS_B_RH_Braking_Cmd_Val1 : Outport  Port=176
  V_BCM_COM_DFCS_A_DBCU_Alt_Mode_1_Val : Outport  Port=177
  V_BCM_COM_DFCS_A_DBCU_Alt_Mode_2_Val : Outport  Port=178
  V_BCM_COM_DFCS_B_DBCU_Alt_Mode_1_Val : Outport  Port=179
  V_BCM_COM_DFCS_B_DBCU_Alt_Mode_2_Val : Outport  Port=180
  V_BCM_COM_DFCS_A_TLA_Above_Idle_Val1 : Outport  Port=181
  V_BCM_COM_DFCS_B_TLA_Above_Idle_Val1 : Outport  Port=182
  V_BCM_COM_UTC_Time_Hours_Cons : Outport  Port=183
  V_BCM_COM_UTC_Time_Hours_Cons_Val : Outport  Port=184
  V_BCM_COM_UTC_Time_Minutes_Cons : Outport  Port=185
  V_BCM_COM_UTC_Time_Minutes_Cons_Val : Outport  Port=186
  V_BCM_COM_UTC_Time_Seconds_Cons : Outport  Port=187
  V_BCM_COM_UTC_Time_Seconds_Cons_Val : Outport  Port=188
  V_BCM_COM_DBCU_BRK_ORDER_FAIL_Conf : Outport  Port=189
  V_BCM_COM_DBCU_DISPATCH_SW_ON_Conf : Outport  Port=190
  V_BCM_COM_LH_DBCU_BRK_CMD_FDBK_Conf : Outport  Port=191
  V_BCM_COM_RH_DBCU_BRK_CMD_FDBK_Conf : Outport  Port=192
  V_BCM_COM_DBCU_FAILED_Conf : Outport  Port=193
  V_BCM_COM_DBCU_ALT_MODE_Conf : Outport  Port=194
  V_BCM_COM_DBCU_BRK_ORDER_FAIL_Cons : Outport  Port=195
  V_BCM_COM_DBCU_BRK_ORDER_FAIL_Cons_Val : Outport  Port=196
  V_BCM_COM_DBCU_DISPATCH_SW_ON_Cons : Outport  Port=197
  V_BCM_COM_DBCU_DISPATCH_SW_ON_Cons_Val : Outport  Port=198
  V_BCM_COM_LH_DBCU_BRK_CMD_FDBK_Cons : Outport  Port=199
  V_BCM_COM_LH_DBCU_BRK_CMD_FDBK_Cons_Val : Outport  Port=200
  V_BCM_COM_RH_DBCU_BRK_CMD_FDBK_Cons : Outport  Port=201
  V_BCM_COM_RH_DBCU_BRK_CMD_FDBK_Cons_Val : Outport  Port=202
  V_BCM_COM_DBCU_FAILED_Cons : Outport  Port=203
  V_BCM_COM_DBCU_FAILED_Cons_Val : Outport  Port=204
  V_BCM_COM_DBCU_ALT_MODE_Cons : Outport  Port=205
  V_BCM_COM_DBCU_ALT_MODE_Cons_Val : Outport  Port=206
  V_BCM_COM_ACCU_PT_Cons : Outport  Port=207
  V_BCM_COM_ACCU_PT_Cons_Val : Outport  Port=208
  V_BCM_COM_ACCU_Pressure_State : Outport  Port=209
  V_BCM_COM_LH_Brake_Temp_Cons : Outport  Port=210
  V_BCM_COM_LH_Brake_Temp_Cons_Val : Outport  Port=211
  V_BCM_COM_RH_Brake_Temp_Cons : Outport  Port=212
  V_BCM_COM_RH_Brake_Temp_Cons_Val : Outport  Port=213
  V_BCM_COM_BCP_PARK_OFF_SW_CMD_Conf : Outport  Port=214
  V_BCM_COM_Park_Sw_Cmd_Cons : Outport  Port=215
  V_BCM_COM_Park_Sw_Cmd_Cons_Val : Outport  Port=216
  V_BCM_COM_MP_MAINT_MODE_CMD_28V_Conf : Outport  Port=217
  V_BCM_COM_MP_MAINT_MODE_CMD_GND_Conf : Outport  Port=218
  V_BCM_COM_Maint_Mode_State_Cons : Outport  Port=219
  V_BCM_COM_LNLG_Tire_Press_Cons : Outport  Port=220
  V_BCM_COM_RNLG_Tire_Press_Cons : Outport  Port=221
  V_BCM_COM_LNLG_Tire_Press_Cons_Val : Outport  Port=222
  V_BCM_COM_RNLG_Tire_Press_Cons_Val : Outport  Port=223
  V_BCM_COM_LMLG_Outboard_Tire_Press_Cons : Outport  Port=224
  V_BCM_COM_LMLG_Outboard_Tire_Press_Cons_Val : Outport  Port=225
  V_BCM_COM_LMLG_Inboard_Tire_Press_Cons : Outport  Port=226
  V_BCM_COM_LMLG_Inboard_Tire_Press_Cons_Val : Outport  Port=227
  V_BCM_COM_RMLG_Inboard_Tire_Press_Cons : Outport  Port=228
  V_BCM_COM_RMLG_Inboard_Tire_Press_Cons_Val : Outport  Port=229
  V_BCM_COM_RMLG_Outboard_Tire_Press_Cons : Outport  Port=230
  V_BCM_COM_RMLG_Outboard_Tire_Press_Cons_Val : Outport  Port=231
  V_BCM_COM_A429_SSM_Avionics_Label_005 : Outport  Port=232
  V_BCM_COM_A429_SSM_Avionics_Label_006 : Outport  Port=233
  V_BCM_COM_A429_SSM_Avionics_Label_021 : Outport  Port=234
  V_BCM_COM_A429_SSM_Avionics_Label_022 : Outport  Port=235
  V_BCM_COM_A429_SSM_Avionics_Label_030 : Outport  Port=236
  V_BCM_COM_A429_SSM_Avionics_Label_031 : Outport  Port=237
  V_BCM_COM_A429_SSM_Avionics_Label_032 : Outport  Port=238
  V_BCM_COM_A429_SSM_Avionics_Label_033 : Outport  Port=239
  V_BCM_COM_A429_SSM_Avionics_Label_040 : Outport  Port=240
  V_BCM_COM_A429_SSM_Avionics_Label_041 : Outport  Port=241
  V_BCM_COM_A429_SSM_Avionics_Label_042 : Outport  Port=242
  V_BCM_COM_A429_SSM_Avionics_Label_043 : Outport  Port=243
  V_BCM_COM_A429_SSM_Avionics_Label_050 : Outport  Port=244
  V_BCM_COM_A429_SSM_DFCS_Label_105 : Outport  Port=245
  V_BCM_COM_A429_Wheel_Speed_W12 : Outport  Port=246
  V_BCM_COM_A429_Wheel_Speed_W34 : Outport  Port=247
  V_BCM_COM_A429_TACHO_Fail_W12 : Outport  Port=248
  V_BCM_COM_A429_TACHO_Fail_W34 : Outport  Port=249
  V_BCM_COM_A429_SSM_Avionics_Label_001 : Outport  Port=250
  V_BCM_COM_A429_SSM_Avionics_Label_002 : Outport  Port=251
  V_BCM_COM_A429_SSM_Avionics_Label_003 : Outport  Port=252
  V_BCM_COM_A429_SSM_Avionics_Label_004 : Outport  Port=253
  V_BCM_COM_A429_SSM_DFCS_Label_101 : Outport  Port=254
  V_BCM_COM_A429_SSM_DFCS_Label_102 : Outport  Port=255
  V_BCM_COM_A429_SSM_DFCS_Label_103 : Outport  Port=256
  V_BCM_COM_A429_SSM_DFCS_Label_104 : Outport  Port=257
  V_BCM_COM_A429_LH_Brake_Temp : Outport  Port=258
  V_BCM_COM_A429_RH_Brake_Temp : Outport  Port=259
  V_BCM_COM_A429_LH_Brake_Temp_Sensor_Fail : Outport  Port=260
  V_BCM_COM_A429_RH_Brake_Temp_Sensor_Fail : Outport  Port=261
  V_BCM_COM_A429_SSM_Avionics_Label_010 : Outport  Port=262
  V_BCM_COM_A429_SSM_Avionics_Label_011 : Outport  Port=263
  V_BCM_COM_A429_LNLG_Tire_Press : Outport  Port=264
  V_BCM_COM_A429_RNLG_Tire_Press : Outport  Port=265
  V_BCM_COM_A429_LMLG_Outboard_Tire_Press : Outport  Port=266
  V_BCM_COM_A429_LMLG_Inboard_Tire_Press : Outport  Port=267
  V_BCM_COM_A429_RMLG_Inboard_Tire_Press : Outport  Port=268
  V_BCM_COM_A429_RMLG_Outboard_Tire_Press : Outport  Port=269
  V_BCM_COM_A429_LNLG_Tire_Press_Sensor_Fail : Outport  Port=270
  V_BCM_COM_A429_RNLG_Tire_Press_Sensor_Fail : Outport  Port=271
  V_BCM_COM_A429_LMLG_Outboard_Tire_Press_Sensor_Fail : Outport  Port=272
  V_BCM_COM_A429_LMLG_Inboard_Tire_Press_Sensor_Fail : Outport  Port=273
  V_BCM_COM_A429_RMLG_Inboard_Tire_Press_Sensor_Fail : Outport  Port=274
  V_BCM_COM_A429_RMLG_Outboard_Tire_Press_Sensor_Fail : Outport  Port=275
  V_BCM_COM_A429_TPIS_Fail : Outport  Port=276
  V_BCM_COM_A429_SSM_Avionics_Label_012 : Outport  Port=277
  V_BCM_COM_A429_SSM_Avionics_Label_013 : Outport  Port=278
  V_BCM_COM_A429_SSM_Avionics_Label_014 : Outport  Port=279
  V_BCM_COM_A429_SSM_Avionics_Label_015 : Outport  Port=280
  V_BCM_COM_A429_SSM_Avionics_Label_016 : Outport  Port=281
  V_BCM_COM_A429_SSM_Avionics_Label_017 : Outport  Port=282
  V_BCM_COM_A429_Curr_Ord_Before_AS : Outport  Port=283
  V_BCM_COM_A429_AS_Curr_Order : Outport  Port=284
  V_BCM_COM_A429_SV_Current_Readback : Outport  Port=285
  V_BCM_COM_A429_SV_PT_In_Bar : Outport  Port=286
  V_BCM_COM_A429_SV_PT_In_PSI : Outport  Port=287
  V_BCM_COM_A429_Antiskid_Activity : Outport  Port=288
  V_BCM_COM_A429_ACCU_PT_Fail : Outport  Port=289
  V_BCM_COM_A429_SV_PT_Fail : Outport  Port=290
  V_BCM_COM_A429_SV_Fail : Outport  Port=291
  V_BCM_COM_A429_ACCU_PT : Outport  Port=292
  V_BCM_COM_A429_SELV_Disc_Sts_Rdbk : Outport  Port=293
  V_BCM_COM_A429_SELV_Disc_Sts_Rdbk_Val : Outport  Port=294
  V_BCM_COM_A429_SELV_Fail : Outport  Port=295
  V_BCM_COM_A429_SSM_Avionics_Label_020 : Outport  Port=296
  V_BCM_COM_A429_SSM_Avionics_Label_036 : Outport  Port=297
  V_BCM_COM_A429_SSM_Avionics_Label_037 : Outport  Port=298
  V_BCM_COM_A429_SSM_DFCS_Label_106 : Outport  Port=299
  V_BCM_COM_A429_SSM_DFCS_Label_107 : Outport  Port=300
  V_BCM_COM_A429_SSM_Avionics_Label_034 : Outport  Port=301
  V_BCM_COM_A429_SSM_Avionics_Label_035 : Outport  Port=302
  V_BCM_COM_A429_Park_Brake_ON : Outport  Port=303
  V_BCM_COM_A429_Park_Brake_Fail : Outport  Port=304
  V_BCM_COM_A429_Norm_FT_In_Progress : Outport  Port=305
  V_BCM_COM_A429_Alt_FT_In_Progress : Outport  Port=306
  V_BCM_COM_A429_Alt_FT_DFCS_Brkg_Req : Outport  Port=307
  V_BCM_COM_A429_Brk_Residual_Press : Outport  Port=308
  V_BCM_COM_A429_PLT_Not_Performed : Outport  Port=309
  V_BCM_COM_A429_Avionics_Comm_Fail_RX : Outport  Port=310
  V_BCM_COM_A429_DFCS_Decel_Law_Inhib : Outport  Port=311
  V_BCM_COM_A429_LH_Brkg_Cmd_Fdbk : Outport  Port=312
  V_BCM_COM_A429_RH_Brkg_Cmd_Fdbk : Outport  Port=313
  V_BCM_COM_A429_DFCS_LH_Brk_Pdl_Ord_Fail : Outport  Port=314
  V_BCM_COM_A429_DFCS_RH_Brk_Pdl_Ord_Fail : Outport  Port=315
  V_BCM_COM_A429_DFCS_A_Comm_Fail_RX : Outport  Port=316
  V_BCM_COM_A429_DFCS_B_Comm_Fail_RX : Outport  Port=317
  V_BCM_COM_A429_DFCS_A_Capsule_Fail : Outport  Port=318
  V_BCM_COM_A429_DFCS_B_Capsule_Fail : Outport  Port=319
  V_BCM_COM_A429_Pinprog_1 : Outport  Port=320
  V_BCM_COM_A429_Pinprog_2 : Outport  Port=321
  V_BCM_COM_A429_Pinprog_3 : Outport  Port=322
  V_BCM_COM_A429_Pinprog_4 : Outport  Port=323
  V_BCM_COM_A429_Pinprog_5 : Outport  Port=324
  V_BCM_COM_A429_PP_Channel_ID : Outport  Port=325
  V_BCM_COM_A429_DBCU_Dispatch_Conf : Outport  Port=326
  V_BCM_COM_A429_Maint_Mode_Active : Outport  Port=327
  V_BCM_COM_A429_Maint_Mode_Req_GND : Outport  Port=328
  V_BCM_COM_A429_Maint_Mode_Req_28V : Outport  Port=329
  V_BCM_COM_A429_Pinprog_Fail : Outport  Port=330
  V_BCM_COM_A429_Norm_Brake_Fail : Outport  Port=331
  V_BCM_COM_A429_BCM_Passivated : Outport  Port=332
  V_BCM_COM_A429_BCM_Fail : Outport  Port=333
  V_BCM_COM_A429_DBCU_Fail : Outport  Port=334
  V_BCM_COM_A429_Alternate_Fail : Outport  Port=335
  V_BCM_COM_A429_DBCU_LH_Brk_Cmd_Fdbk : Outport  Port=336
  V_BCM_COM_A429_DBCU_RH_Brk_Cmd_Fdbk : Outport  Port=337
  V_BCM_COM_A429_DBCU_Inhib_Opp_Side : Outport  Port=338
  V_BCM_COM_A429_DBCU_Alt_Mode : Outport  Port=339
  V_BCM_COM_A429_SSM_DFCS_Label_100 : Outport  Port=340
  V_BCM_COM_A429_Global_Wheel_Spd : Outport  Port=341
  V_BCM_COM_ETH_HYD_A_PRESS : Outport  Port=342
  V_BCM_COM_ETH_HYD_B_PRESS : Outport  Port=343
  V_BCM_COM_ETH_ENG1_RUNNING : Outport  Port=344
  V_BCM_COM_ETH_ENG2_RUNNING : Outport  Port=345
  V_BCM_COM_ETH_LMLG_Dnlk : Outport  Port=346
  V_BCM_COM_ETH_RMLG_Dnlk : Outport  Port=347
  V_BCM_COM_ETH_Lever_Up : Outport  Port=348
  V_BCM_COM_ETH_BCP_BCM_ALT_SW_ON_CMD : Outport  Port=349
  V_BCM_COM_ETH_MP_MAINT_MODE_CMD_GND : Outport  Port=350
  V_BCM_COM_ETH_MP_MAINT_MODE_CMD_28V : Outport  Port=351
  V_BCM_COM_ETH_MP_BCMA_ALT_DISP_SW : Outport  Port=352
  V_BCM_COM_ETH_PBSELV_ON_POS : Outport  Port=353
  V_BCM_COM_ETH_DBCU_BRK_ORDER_FAIL : Outport  Port=354
  V_BCM_COM_ETH_DISPATCH_SW_ON : Outport  Port=355
  V_BCM_COM_ETH_LH_DBCU_BRK_CMD_FDBK : Outport  Port=356
  V_BCM_COM_ETH_RH_DBCU_BRK_CMD_FDBK : Outport  Port=357
  V_BCM_COM_ETH_DBCU_FAILED : Outport  Port=358
  V_BCM_COM_ETH_ALT_MODE : Outport  Port=359
  V_BCM_COM_ETH_Opp_BCM_DBCU_INHIB : Outport  Port=360
  V_BCM_COM_ETH_LH_SV_Current_Order : Outport  Port=361
  V_BCM_COM_ETH_RH_SV_Current_Order : Outport  Port=362
  V_BCM_COM_ETH_SELV_High_Side_Cmd_Order : Outport  Port=363
  V_BCM_COM_ETH_DBCU_Inhib_Order : Outport  Port=364
  V_BCM_COM_ETH_FB_BCM_FAIL : Outport  Port=365
  V_BCM_COM_ETH_FB_DFCS_A_RX : Outport  Port=366
  V_BCM_COM_ETH_FB_DFCS_B_RX : Outport  Port=367
  V_BCM_COM_ETH_FB_MAINT_MODE_DIS : Outport  Port=368
  V_BCM_COM_ETH_FB_PARK_BRK_STATUS_DIS : Outport  Port=369
  V_BCM_COM_ETH_FB_BCM_DBCU_MODE_DIS : Outport  Port=370
  V_BCM_COM_ETH_FB_DBCU_SIMULT_ACT : Outport  Port=371
  V_BCM_COM_ETH_FB_DBCU_FAIL : Outport  Port=372
  V_BCM_COM_ETH_FB_DBCU_BRK_ORDER_FAIL : Outport  Port=373
  V_BCM_COM_ETH_FB_INHIB_FAIL : Outport  Port=374
  V_BCM_COM_ETH_FB_HYD_A_LOW_PRESS : Outport  Port=375
  V_BCM_COM_ETH_FB_HYD_B_LOW_PRESS : Outport  Port=376
  V_BCM_COM_ETH_FB_ACCU_LOW_PRESS : Outport  Port=377
  V_BCM_COM_ETH_FB_ACCU_PT_FAIL : Outport  Port=378
  V_BCM_COM_ETH_FB_BSELV_CMD_FAIL : Outport  Port=379
  V_BCM_COM_ETH_FB_BSELV_JCL : Outport  Port=380
  V_BCM_COM_ETH_FB_BSELV_JOP : Outport  Port=381
  V_BCM_COM_ETH_FB_LH_SV_PT_FAIL : Outport  Port=382
  V_BCM_COM_ETH_FB_LH_SV_CMD_FAIL : Outport  Port=383
  V_BCM_COM_ETH_FB_LH_SV_JCL : Outport  Port=384
  V_BCM_COM_ETH_FB_LH_SV_JOP : Outport  Port=385
  V_BCM_COM_ETH_FB_RH_SV_PT_FAIL : Outport  Port=386
  V_BCM_COM_ETH_FB_RH_SV_CMD_FAIL : Outport  Port=387
  V_BCM_COM_ETH_FB_RH_SV_JCL : Outport  Port=388
  V_BCM_COM_ETH_FB_RH_SV_JOP : Outport  Port=389
  V_BCM_COM_ETH_AC_State : Outport  Port=390
  V_BCM_COM_ETH_AC_Flight_Phase : Outport  Port=391
  V_BCM_COM_ETH_Braking_Mode : Outport  Port=392
  V_BCM_COM_ETH_Braking_Norm_FT_Seq : Outport  Port=393
  V_BCM_COM_ETH_Braking_Alt_FT_Seq : Outport  Port=394
  V_BCM_COM_ETH_FB_LG_LEVER_FAIL : Outport  Port=395
  V_BCM_COM_ETH_FB_LMLG_DWNLOCK_FAIL : Outport  Port=396
  V_BCM_COM_ETH_FB_RMLG_DWNLOCK_FAIL : Outport  Port=397
  V_BCM_COM_ETH_TARGET_HW_ID : Outport  Port=398
  V_BCM_COM_ETH_Invalid_Config : Outport  Port=399
  V_BCM_COM_ETH_FB_LH_OUT_TACHO_FAIL : Outport  Port=400
  V_BCM_COM_ETH_FB_LH_IN_TACHO_FAIL : Outport  Port=401
  V_BCM_COM_ETH_FB_RH_IN_TACHO_FAIL : Outport  Port=402
  V_BCM_COM_ETH_FB_RH_OUT_TACHO_FAIL : Outport  Port=403
  V_BCM_COM_ETH_TT_in_progress_id : Outport  Port=404
  V_BCM_COM_ETH_TT_rejection_cause : Outport  Port=405
  V_BCM_COM_ETH_TT_rejected : Outport  Port=406
  V_BCM_COM_ETH_TT_completed : Outport  Port=407
  V_BCM_COM_ETH_TT_result_significant : Outport  Port=408
  V_BCM_COM_BCM_DBCU_INHIBITION_Conf : Outport  Port=409
  V_BCM_COM_Target_DCL : Outport  Port=410
  V_BCM_COM_Decel_Ctrl_Loop_Act_Cond : Outport  Port=411
  wires:
  V_BCM_COM_Tachometers_Conf_Flt/1 -> Selector1/1, Selector/1
  V_BCM_COM_DFCS_B_Gnd_Spd_Acq/1 -> BCM_COM_PROC_P20/4(V_BCM_COM_DFCS_B_Gnd_Spd_Acq)
  V_BCM_COM_DFCS_A_Gnd_Spd_Acq/1 -> BCM_COM_PROC_P20/3(V_BCM_COM_DFCS_A_Gnd_Spd_Acq)
  V_BCM_COM_DFCS_B_Long_Accel_Acq/1 -> BCM_COM_PROC_P20/6(V_BCM_COM_DFCS_B_Long_Accel_Acq)
  V_BCM_COM_DFCS_A_Long_Accel_Acq/1 -> BCM_COM_PROC_P20/5(V_BCM_COM_DFCS_A_Long_Accel_Acq)
  V_BCM_COM_DFCS_B_Pitch_Ang_Acq/1 -> BCM_COM_PROC_P20/8(V_BCM_COM_DFCS_B_Pitch_Ang_Acq)
  V_BCM_COM_DFCS_A_Pitch_Ang_Acq/1 -> BCM_COM_PROC_P20/7(V_BCM_COM_DFCS_A_Pitch_Ang_Acq)
  V_BCM_COM_DFCS_B_LMLG_WOWs_Acq/1 -> BCM_COM_PROC_P20/10(V_BCM_COM_DFCS_B_LMLG_WOWs_Acq)
  V_BCM_COM_DFCS_A_LMLG_WOWs_Acq/1 -> BCM_COM_PROC_P20/9(V_BCM_COM_DFCS_A_LMLG_WOWs_Acq)
  V_BCM_COM_DFCS_A_RMLG_WOWs_Acq/1 -> BCM_COM_PROC_P20/11(V_BCM_COM_DFCS_A_RMLG_WOWs_Acq)
  V_BCM_COM_DFCS_B_RMLG_WOWs_Acq/1 -> BCM_COM_PROC_P20/12(V_BCM_COM_DFCS_B_RMLG_WOWs_Acq)
  V_BCM_COM_DFCS_A_NLG_WOWs_Acq/1 -> BCM_COM_PROC_P20/13(V_BCM_COM_DFCS_A_NLG_WOWs_Acq)
  V_BCM_COM_DFCS_B_NLG_WOWs_Acq/1 -> BCM_COM_PROC_P20/14(V_BCM_COM_DFCS_B_NLG_WOWs_Acq)
  V_BCM_COM_DFCS_B_WOWs_Val_Acq/1 -> BCM_COM_PROC_P20/16(V_BCM_COM_DFCS_B_WOWs_Val_Acq)
  V_BCM_COM_DFCS_A_WOWs_Val_Acq/1 -> BCM_COM_PROC_P20/15(V_BCM_COM_DFCS_A_WOWs_Val_Acq)
  V_BCM_COM_RH_Decel_Law_Brkg_Press_Cmd/1 -> BCM_COM_PROC_P20/17(V_BCM_COM_RH_Decel_Law_Brkg_Press_Cmd)
  V_BCM_COM_LH_Decel_Law_Brkg_Press_Cmd/1 -> BCM_COM_PROC_P20/18(V_BCM_COM_LH_Decel_Law_Brkg_Press_Cmd)
  V_BCM_COM_DFCS_A_DFCS_RH_Braking_Cmd_Acq/1 -> BCM_COM_PROC_P20/20(V_BCM_COM_DFCS_A_DFCS_RH_Braking_Cmd_Acq)
  V_BCM_COM_DFCS_A_DFCS_LH_Braking_Cmd_Acq/1 -> BCM_COM_PROC_P20/19(V_BCM_COM_DFCS_A_DFCS_LH_Braking_Cmd_Acq)
  V_BCM_COM_DFCS_B_DFCS_RH_Braking_Cmd_Acq/1 -> BCM_COM_PROC_P20/22(V_BCM_COM_DFCS_B_DFCS_RH_Braking_Cmd_Acq)
  V_BCM_COM_DFCS_B_DFCS_LH_Braking_Cmd_Acq/1 -> BCM_COM_PROC_P20/21(V_BCM_COM_DFCS_B_DFCS_LH_Braking_Cmd_Acq)
  V_BCM_COM_DFCS_A_Decel_Law_Inhib_Acq/1 -> BCM_COM_PROC_P20/23(V_BCM_COM_DFCS_A_Decel_Law_Inhib_Acq)
  V_BCM_COM_DFCS_B_Decel_Law_Inhib_Acq/1 -> BCM_COM_PROC_P20/24(V_BCM_COM_DFCS_B_Decel_Law_Inhib_Acq)
  V_BCM_COM_DFCS_A_TLA_Above_Idle_Acq/1 -> BCM_COM_PROC_P20/25(V_BCM_COM_DFCS_A_TLA_Above_Idle_Acq)
  V_BCM_COM_DFCS_B_TLA_Above_Idle_Acq/1 -> BCM_COM_PROC_P20/26(V_BCM_COM_DFCS_B_TLA_Above_Idle_Acq)
  V_BCM_COM_LG_Lever_Up_Acq/1 -> BCM_COM_PROC_P20/27(V_BCM_COM_LG_Lever_Up_Acq)
  V_BCM_COM_LG_Lever_Up_Unconf_Flt/1 -> BCM_COM_PROC_P20/28(V_BCM_COM_LG_Lever_Up_Unconf_Flt)
  V_BCM_COM_LG_Lever_Up_Conf_Flt/1 -> BCM_COM_PROC_P20/29(V_BCM_COM_LG_Lever_Up_Conf_Flt)
  V_BCM_COM_LMLG_Downlock_Acq/1 -> BCM_COM_PROC_P20/30(V_BCM_COM_LMLG_Downlock_Acq)
  V_BCM_COM_RMLG_Downlock_Acq/1 -> BCM_COM_PROC_P20/31(V_BCM_COM_RMLG_Downlock_Acq)
  V_BCM_COM_LMLG_Dnlk_Unconf_Flt/1 -> BCM_COM_PROC_P20/32(V_BCM_COM_LMLG_Dnlk_Unconf_Flt)
  V_BCM_COM_LMLG_Dnlk_Conf_Flt/1 -> BCM_COM_PROC_P20/33(V_BCM_COM_LMLG_Dnlk_Conf_Flt)
  V_BCM_COM_RMLG_Dnlk_Conf_Flt/1 -> BCM_COM_PROC_P20/35(V_BCM_COM_RMLG_Dnlk_Conf_Flt)
  V_BCM_COM_RMLG_Dnlk_Unconf_Flt/1 -> BCM_COM_PROC_P20/34(V_BCM_COM_RMLG_Dnlk_Unconf_Flt)
  V_BCM_COM_Engine_Running_Acq/1 -> BCM_COM_PROC_P20/36(V_BCM_COM_Engine_Running_Acq)
  V_BCM_COM_Maint_Itv_Function_Req/1 -> BCM_COM_PROC_P20/37(V_BCM_COM_Maint_Itv_Function_Req)
  V_BCM_COM_BCM_Config/1 -> BCM_COM_PROC_P20/38(V_BCM_COM_BCM_Config)
  V_BCM_COM_Hyd_B_Press_Acq/1 -> BCM_COM_PROC_P20/57(V_BCM_COM_Hyd_B_Press_Acq)
  V_BCM_COM_PBSELV_ON_POS_Acq/1 -> BCM_COM_PROC_P20/53(V_BCM_COM_PBSELV_ON_POS_Acq)
  V_BCM_COM_SV_PT_Filt/1 -> BCM_COM_PROC_P20/52(V_BCM_COM_SV_PT_Filt)
  V_BCM_COM_BCM_Off_Sanction/1 -> BCM_COM_PROC_P20/39(V_BCM_COM_BCM_Off_Sanction)
  V_BCM_COM_BCM_Validity_By_SP/1 -> BCM_COM_PROC_P20/40(V_BCM_COM_BCM_Validity_By_SP)
  V_BCM_COM_BCP_BCM_Alt_Sw_On_Cmd_Acq/1 -> BCM_COM_PROC_P20/41(V_BCM_COM_BCP_BCM_Alt_Sw_On_Cmd_Acq)
  V_BCM_COM_BCP_BCM_Alt_Sw_On_Cmd_Conf_Flt/1 -> BCM_COM_PROC_P20/42(V_BCM_COM_BCP_BCM_Alt_Sw_On_Cmd_Conf_Flt)
  V_BCM_COM_BCP_BCM_Alt_Sw_On_Cmd_Unconf_Flt/1 -> BCM_COM_PROC_P20/43(V_BCM_COM_BCP_BCM_Alt_Sw_On_Cmd_Unconf_Flt)
  V_BCM_COM_MP_BCMA_Alt_Disp_Sw_Conf_Flt/1 -> BCM_COM_PROC_P20/44(V_BCM_COM_MP_BCMA_Alt_Disp_Sw_Conf_Flt)
  V_BCM_COM_MP_BCMA_Alt_Disp_Sw_Unconf_Flt/1 -> BCM_COM_PROC_P20/45(V_BCM_COM_MP_BCMA_Alt_Disp_Sw_Unconf_Flt)
  V_BCM_COM_MP_BCMA_Alt_Disp_Sw_Acq/1 -> BCM_COM_PROC_P20/46(V_BCM_COM_MP_BCMA_Alt_Disp_Sw_Acq)
  V_BCM_COM_Antiskid_Off_Sanction/1 -> BCM_COM_PROC_P20/47(V_BCM_COM_Antiskid_Off_Sanction)
  V_BCM_COM_Norm_Brkg_Off_Sanc/1 -> BCM_COM_PROC_P20/48(V_BCM_COM_Norm_Brkg_Off_Sanc)
  V_BCM_COM_CF_LH_ALT_BRK_LOSS/1 -> BCM_COM_PROC_P20/49(V_BCM_COM_CF_LH_ALT_BRK_LOSS)
  V_BCM_COM_CF_DBCU_FAILED/1 -> BCM_COM_PROC_P20/50(V_BCM_COM_CF_DBCU_FAILED)
  V_BCM_COM_CF_RH_ALT_BRK_LOSS/1 -> BCM_COM_PROC_P20/51(V_BCM_COM_CF_RH_ALT_BRK_LOSS)
  V_BCM_COM_PBSELV_ON_POS_Unconf_Flt/1 -> BCM_COM_PROC_P20/54(V_BCM_COM_PBSELV_ON_POS_Unconf_Flt)
  V_BCM_COM_Hyd_A_Press_Acq/1 -> BCM_COM_PROC_P20/56(V_BCM_COM_Hyd_A_Press_Acq)
  V_BCM_COM_PBSELV_ON_POS_Conf_Flt/1 -> BCM_COM_PROC_P20/55(V_BCM_COM_PBSELV_ON_POS_Conf_Flt)
  V_BCM_COM_Whl_AS_Inhib_Cond_W12/1 -> BCM_COM_PROC_P20/58(V_BCM_COM_Whl_AS_Inhib_Cond_W12)
  V_BCM_COM_Whl_AS_Inhib_Cond_W34/1 -> BCM_COM_PROC_P20/59(V_BCM_COM_Whl_AS_Inhib_Cond_W34)
  V_BCM_COM_Whl_LP_AS_Curr_Order/1 -> BCM_COM_PROC_P20/60(V_BCM_COM_Whl_LP_AS_Curr_Order)
  V_BCM_COM_SV_PT_Cons/1 -> BCM_COM_PROC_P20/61(V_BCM_COM_SV_PT_Cons)
  V_BCM_COM_Wheel_Filtered_Speed_W12/1 -> BCM_COM_PROC_P20/62(V_BCM_COM_Wheel_Filtered_Speed_W12)
  V_BCM_COM_Wheel_Filtered_Speed_W34/1 -> BCM_COM_PROC_P20/63(V_BCM_COM_Wheel_Filtered_Speed_W34)
  V_BCM_COM_Wheel_Speed_Error_W12/1 -> BCM_COM_PROC_P20/64(V_BCM_COM_Wheel_Speed_Error_W12)
  V_BCM_COM_Wheel_Speed_Error_W34/1 -> BCM_COM_PROC_P20/65(V_BCM_COM_Wheel_Speed_Error_W34)
  V_BCM_COM_Whl_LP_AS_Curr_Order_W12/1 -> BCM_COM_PROC_P20/66(V_BCM_COM_Whl_LP_AS_Curr_Order_W12)
  V_BCM_COM_Whl_LP_AS_Curr_Order_W34/1 -> BCM_COM_PROC_P20/67(V_BCM_COM_Whl_LP_AS_Curr_Order_W34)
  V_BCM_COM_SV_Current/1 -> BCM_COM_PROC_P20/68(V_BCM_COM_SV_Current)
  V_BCM_COM_SV_PT_Cons_Val/1 -> BCM_COM_PROC_P20/69(V_BCM_COM_SV_PT_Cons_Val)
  V_BCM_COM_Opt_Adhesion_In_Acq_W12/1 -> BCM_COM_PROC_P20/74(V_BCM_COM_Opt_Adhesion_In_Acq_W12)
  V_BCM_COM_Opt_Adhesion_In_Acq_W34/1 -> BCM_COM_PROC_P20/75(V_BCM_COM_Opt_Adhesion_In_Acq_W34)
  V_BCM_COM_Adhesion_In_Acq_W12/1 -> BCM_COM_PROC_P20/72(V_BCM_COM_Adhesion_In_Acq_W12)
  V_BCM_COM_Adhesion_In_Acq_W34/1 -> BCM_COM_PROC_P20/73(V_BCM_COM_Adhesion_In_Acq_W34)
  V_BCM_COM_Target_Speed_In_Acq_W12/1 -> BCM_COM_PROC_P20/76(V_BCM_COM_Target_Speed_In_Acq_W12)
  V_BCM_COM_Target_Speed_In_Acq_W34/1 -> BCM_COM_PROC_P20/77(V_BCM_COM_Target_Speed_In_Acq_W34)
  V_BCM_COM_Big_Gamma_Trig_In_Acq_W12/1 -> BCM_COM_PROC_P20/80(V_BCM_COM_Big_Gamma_Trig_In_Acq_W12)
  V_BCM_COM_Big_Gamma_Trig_In_Acq_W34/1 -> BCM_COM_PROC_P20/81(V_BCM_COM_Big_Gamma_Trig_In_Acq_W34)
  V_BCM_COM_Small_Slip_Trig_In_Acq_W12/1 -> BCM_COM_PROC_P20/82(V_BCM_COM_Small_Slip_Trig_In_Acq_W12)
  V_BCM_COM_Small_Slip_Trig_In_Acq_W34/1 -> BCM_COM_PROC_P20/83(V_BCM_COM_Small_Slip_Trig_In_Acq_W34)
  V_BCM_COM_Big_Slip_Trig_In_Acq_W12/1 -> BCM_COM_PROC_P20/84(V_BCM_COM_Big_Slip_Trig_In_Acq_W12)
  V_BCM_COM_Big_Slip_Trig_In_Acq_W34/1 -> BCM_COM_PROC_P20/85(V_BCM_COM_Big_Slip_Trig_In_Acq_W34)
  Selector/1 -> BCM_COM_PROC_P20/1(V_BCM_COM_Tacho_Conf_Flt_W12)
  Selector1/1 -> BCM_COM_PROC_P20/2(V_BCM_COM_Tacho_Conf_Flt_W34)
  V_BCM_COM_DFCS_A_Gnd_Spd_Val/1 -> BCM_COM_PROC_P20/93(V_BCM_COM_DFCS_A_Gnd_Spd_Acq_Val)
  V_BCM_COM_DFCS_A_AC_Long_Accel_Val/1 -> BCM_COM_PROC_P20/94(V_BCM_COM_DFCS_A_Long_Accel_Acq_Val)
  V_BCM_COM_DFCS_A_AC_Pitch_Angle_Val/1 -> BCM_COM_PROC_P20/95(V_BCM_COM_DFCS_A_Pitch_Angle_Acq_Val)
  V_BCM_COM_DFCS_A_Decel_Law_Inhib_Val/1 -> BCM_COM_PROC_P20/96(V_BCM_COM_DFCS_A_Decel_Law_Inhib_Acq_Val)
  V_BCM_COM_DFCS_B_Decel_Law_Inhib_Val/1 -> BCM_COM_PROC_P20/97(V_BCM_COM_DFCS_B_Decel_Law_Inhib_Acq_Val)
  V_BCM_COM_DFCS_B_Gnd_Spd_Val/1 -> BCM_COM_PROC_P20/98(V_BCM_COM_DFCS_B_Gnd_Spd_Acq_Val)
  V_BCM_COM_DFCS_B_AC_Long_Accel_Val/1 -> BCM_COM_PROC_P20/99(V_BCM_COM_DFCS_B_Long_Accel_Acq_Val)
  V_BCM_COM_DFCS_B_AC_Pitch_Angle_Val/1 -> BCM_COM_PROC_P20/100(V_BCM_COM_DFCS_B_Pitch_Angle_Acq_Val)
  V_BCM_COM_DFCS_A_LMLG_WOWs_Val/1 -> Demux/1
  Demux/1 -> BCM_COM_PROC_P20/101(V_BCM_COM_DFCS_A_Lmlg_Wow_1_Acq_Val)
  Demux/2 -> BCM_COM_PROC_P20/102(V_BCM_COM_DFCS_A_Lmlg_Wow_2_Acq_Val)
  Demux/3 -> BCM_COM_PROC_P20/103(V_BCM_COM_DFCS_A_Lmlg_Wow_3_Acq_Val)
  V_BCM_COM_DFCS_A_RMLG_WOWs_Val/1 -> Demux1/1
  Demux1/1 -> BCM_COM_PROC_P20/104(V_BCM_COM_DFCS_A_Rmlg_Wow_1_Acq_Val)
  Demux1/2 -> BCM_COM_PROC_P20/105(V_BCM_COM_DFCS_A_Rmlg_Wow_2_Acq_Val)
  Demux1/3 -> BCM_COM_PROC_P20/106(V_BCM_COM_DFCS_A_Rmlg_Wow_3_Acq_Val)
  V_BCM_COM_DFCS_A_NLG_WOWs_Val/1 -> Demux2/1
  Demux2/1 -> BCM_COM_PROC_P20/107(V_BCM_COM_DFCS_A_Nlg_Wow_1_Acq_Val)
  Demux2/2 -> BCM_COM_PROC_P20/108(V_BCM_COM_DFCS_A_Nlg_Wow_2_Acq_Val)
  Demux2/3 -> BCM_COM_PROC_P20/109(V_BCM_COM_DFCS_A_Nlg_Wow_3_Acq_Val)
  V_BCM_COM_DFCS_A_WOWs_Val_Val/1 -> Demux3/1
  Demux3/1 -> BCM_COM_PROC_P20/110(V_BCM_COM_DFCS_A_Wow_Val_1_Acq_Val)
  Demux3/2 -> BCM_COM_PROC_P20/111(V_BCM_COM_DFCS_A_Wow_Val_2_Acq_Val)
  Demux3/3 -> BCM_COM_PROC_P20/112(V_BCM_COM_DFCS_A_Wow_Val_3_Acq_Val)
  Demux4/1 -> BCM_COM_PROC_P20/113(V_BCM_COM_DFCS_B_Lmlg_Wow_1_Acq_Val)
  Demux4/2 -> BCM_COM_PROC_P20/114(V_BCM_COM_DFCS_B_Lmlg_Wow_2_Acq_Val)
  Demux4/3 -> BCM_COM_PROC_P20/115(V_BCM_COM_DFCS_B_Lmlg_Wow_3_Acq_Val)
  V_BCM_COM_DFCS_B_LMLG_WOWs_Val/1 -> Demux4/1
  V_BCM_COM_DFCS_B_RMLG_WOWs_Val/1 -> Demux5/1
  Demux5/1 -> BCM_COM_PROC_P20/116(V_BCM_COM_DFCS_B_Rmlg_Wow_1_Acq_Val)
  Demux5/2 -> BCM_COM_PROC_P20/117(V_BCM_COM_DFCS_B_Rmlg_Wow_2_Acq_Val)
  Demux5/3 -> BCM_COM_PROC_P20/118(V_BCM_COM_DFCS_B_Rmlg_Wow_3_Acq_Val)
  Demux6/3 -> BCM_COM_PROC_P20/121(V_BCM_COM_DFCS_B_Nlg_Wow_3_Acq_Val)
  Demux6/2 -> BCM_COM_PROC_P20/120(V_BCM_COM_DFCS_B_Nlg_Wow_2_Acq_Val)
  Demux6/1 -> BCM_COM_PROC_P20/119(V_BCM_COM_DFCS_B_Nlg_Wow_1_Acq_Val)
  V_BCM_COM_DFCS_B_NLG_WOWs_Val/1 -> Demux6/1
  V_BCM_COM_DFCS_B_WOWs_Val_Val/1 -> Demux7/1
  Demux7/1 -> BCM_COM_PROC_P20/122(V_BCM_COM_DFCS_B_Wow_Val_1_Acq_Val)
  Demux7/2 -> BCM_COM_PROC_P20/123(V_BCM_COM_DFCS_B_Wow_Val_2_Acq_Val)
  Demux7/3 -> BCM_COM_PROC_P20/124(V_BCM_COM_DFCS_B_Wow_Val_3_Acq_Val)
  V_BCM_COM_DFCS_B_RH_Braking_Cmd_Val/1 -> BCM_COM_PROC_P20/125(V_BCM_COM_DFCS_B_DFCS_RH_Brkg_Cmd_Acq_Val)
  V_BCM_COM_DFCS_B_LH_Braking_Cmd_Val/1 -> BCM_COM_PROC_P20/126(V_BCM_COM_DFCS_B_DFCS_LH_Brkg_Cmd_Acq_Val)
  V_BCM_COM_DFCS_A_RH_Braking_Cmd_Val/1 -> BCM_COM_PROC_P20/127(V_BCM_COM_DFCS_A_DFCS_RH_Brkg_Cmd_Acq_Val)
  V_BCM_COM_DFCS_A_LH_Braking_Cmd_Val/1 -> BCM_COM_PROC_P20/128(V_BCM_COM_DFCS_A_DFCS_LH_Brkg_Cmd_Acq_Val)
  V_BCM_COM_DFCS_A_TLA_Above_Idle_Val/1 -> BCM_COM_PROC_P20/133(V_BCM_COM_DFCS_A_TLA_Above_Idle_Acq_Val)
  V_BCM_COM_DFCS_B_TLA_Above_Idle_Val/1 -> BCM_COM_PROC_P20/134(V_BCM_COM_DFCS_B_TLA_Above_Idle_Acq_Val)
  V_BCM_COM_BCM_CCDL_Conf_Flt/1 -> BCM_COM_PROC_P20/70(V_BCM_COM_BCM_CCDL_Conf_Flt)
  V_BCM_COM_BCM_CCDL_Unconf_Flt/1 -> BCM_COM_PROC_P20/71(V_BCM_COM_BCM_CCDL_Unconf_Flt)
  V_BCM_COM_Big_Slip_WD_Trig_In_Acq_W12/1 -> BCM_COM_PROC_P20/78(V_BCM_COM_Big_Slip_WD_Trig_In_Acq_W12)
  V_BCM_COM_Big_Slip_WD_Trig_In_Acq_W34/1 -> BCM_COM_PROC_P20/79(V_BCM_COM_Big_Slip_WD_Trig_In_Acq_W34)
  V_BCM_COM_BCM_DBCU_INHIBITION_Conf_Flt/1 -> BCM_COM_PROC_P20/86(V_BCM_COM_BCM_DBCU_INHIBITION_Conf_Flt)
  V_BCM_COM_BCM_DBCU_INHIBITION_Unconf_Flt/1 -> BCM_COM_PROC_P20/87(V_BCM_COM_BCM_DBCU_INHIBITION_Unconf_Flt)
  V_BCM_COM_BCM_DBCU_INHIBITION_Acq/1 -> BCM_COM_PROC_P20/88(V_BCM_COM_BCM_DBCU_INHIBITION_Acq)
  V_BCM_COM_Engine_1_Running_Acq_Val/1 -> BCM_COM_PROC_P20/89(V_BCM_COM_Engine_1_Running_Acq_Val)
  V_BCM_COM_Engine_2_Running_Acq_Val/1 -> BCM_COM_PROC_P20/90(V_BCM_COM_Engine_2_Running_Acq_Val)
  V_BCM_COM_Hyd_A_Press_Acq_Val/1 -> BCM_COM_PROC_P20/91(V_BCM_COM_Hyd_A_Press_Acq_Val)
  V_BCM_COM_Hyd_B_Press_Acq_Val/1 -> BCM_COM_PROC_P20/92(V_BCM_COM_Hyd_B_Press_Acq_Val)
  V_BCM_COM_DFCS_A_DBCU_ALT_Mode_1_Acq_Val/1 -> BCM_COM_PROC_P20/129(V_BCM_COM_DFCS_A_DBCU_ALT_Mode_1_Acq_Val)
  V_BCM_COM_DFCS_A_DBCU_ALT_Mode_2_Acq_Val/1 -> BCM_COM_PROC_P20/130(V_BCM_COM_DFCS_A_DBCU_ALT_Mode_2_Acq_Val)
  V_BCM_COM_DFCS_B_DBCU_ALT_Mode_1_Acq_Val/1 -> BCM_COM_PROC_P20/131(V_BCM_COM_DFCS_B_DBCU_ALT_Mode_1_Acq_Val)
  V_BCM_COM_DFCS_B_DBCU_ALT_Mode_2_Acq_Val/1 -> BCM_COM_PROC_P20/132(V_BCM_COM_DFCS_B_DBCU_ALT_Mode_2_Acq_Val)
  V_BCM_COM_UTC_Time_Hours_Acq/1 -> BCM_COM_PROC_P20/135(V_BCM_COM_UTC_Time_Hours_Acq)
  V_BCM_COM_UTC_Time_Hours_Conf_Flt/1 -> BCM_COM_PROC_P20/136(V_BCM_COM_UTC_Time_Hours_Conf_Flt)
  V_BCM_COM_UTC_Time_Hours_Unconf_Flt/1 -> BCM_COM_PROC_P20/137(V_BCM_COM_UTC_Time_Hours_Unconf_Flt)
  V_BCM_COM_UTC_Time_Minutes_Acq/1 -> BCM_COM_PROC_P20/138(V_BCM_COM_UTC_Time_Minutes_Acq)
  V_BCM_COM_UTC_Time_Minutes_Conf_Flt/1 -> BCM_COM_PROC_P20/139(V_BCM_COM_UTC_Time_Minutes_Conf_Flt)
  V_BCM_COM_UTC_Time_Minutes_Unconf_Flt/1 -> BCM_COM_PROC_P20/140(V_BCM_COM_UTC_Time_Minutes_Unconf_Flt)
  V_BCM_COM_UTC_Time_Seconds_Acq/1 -> BCM_COM_PROC_P20/141(V_BCM_COM_UTC_Time_Seconds_Acq)
  V_BCM_COM_UTC_Time_Seconds_Conf_Flt/1 -> BCM_COM_PROC_P20/142(V_BCM_COM_UTC_Time_Seconds_Conf_Flt)
  V_BCM_COM_UTC_Time_Seconds_Unconf_Flt/1 -> BCM_COM_PROC_P20/143(V_BCM_COM_UTC_Time_Seconds_Unconf_Flt)
  V_BCM_COM_DBCU_BRK_ORDER_FAIL_Acq/1 -> BCM_COM_PROC_P20/144(V_BCM_COM_DBCU_BRK_ORDER_FAIL_Acq)
  V_BCM_COM_DBCU_DISPATCH_SW_ON_Acq/1 -> BCM_COM_PROC_P20/145(V_BCM_COM_DBCU_DISPATCH_SW_ON_Acq)
  V_BCM_COM_LH_DBCU_BRK_CMD_FDBK_Acq/1 -> BCM_COM_PROC_P20/146(V_BCM_COM_LH_DBCU_BRK_CMD_FDBK_Acq)
  V_BCM_COM_RH_DBCU_BRK_CMD_FDBK_Acq/1 -> BCM_COM_PROC_P20/147(V_BCM_COM_RH_DBCU_BRK_CMD_FDBK_Acq)
  V_BCM_COM_DBCU_FAILED_Acq/1 -> BCM_COM_PROC_P20/148(V_BCM_COM_DBCU_FAILED_Acq)
  V_BCM_COM_DBCU_ALT_MODE_Acq/1 -> BCM_COM_PROC_P20/149(V_BCM_COM_DBCU_ALT_MODE_Acq)
  V_BCM_COM_DBCU_BRK_ORDER_FAIL_Conf_Flt/1 -> BCM_COM_PROC_P20/150(V_BCM_COM_DBCU_BRK_ORDER_FAIL_Conf_Flt)
  V_BCM_COM_DBCU_BRK_ORDER_FAIL_Unconf_Flt/1 -> BCM_COM_PROC_P20/151(V_BCM_COM_DBCU_BRK_ORDER_FAIL_Unconf_Flt)
  V_BCM_COM_DBCU_DISPATCH_SW_ON_Conf_Flt/1 -> BCM_COM_PROC_P20/152(V_BCM_COM_DBCU_DISPATCH_SW_ON_Conf_Flt)
  V_BCM_COM_DBCU_DISPATCH_SW_ON_Unconf_Flt/1 -> BCM_COM_PROC_P20/153(V_BCM_COM_DBCU_DISPATCH_SW_ON_Unconf_Flt)
  V_BCM_COM_LH_DBCU_BRK_CMD_FDBK_Conf_Flt/1 -> BCM_COM_PROC_P20/154(V_BCM_COM_LH_DBCU_BRK_CMD_FDBK_Conf_Flt)
  V_BCM_COM_LH_DBCU_BRK_CMD_FDBK_Unconf_Flt/1 -> BCM_COM_PROC_P20/155(V_BCM_COM_LH_DBCU_BRK_CMD_FDBK_Unconf_Flt)
  V_BCM_COM_RH_DBCU_BRK_CMD_FDBK_Conf_Flt/1 -> BCM_COM_PROC_P20/156(V_BCM_COM_RH_DBCU_BRK_CMD_FDBK_Conf_Flt)
  V_BCM_COM_RH_DBCU_BRK_CMD_FDBK_Unconf_Flt/1 -> BCM_COM_PROC_P20/157(V_BCM_COM_RH_DBCU_BRK_CMD_FDBK_Unconf_Flt)
  V_BCM_COM_DBCU_FAILED_Conf_Flt/1 -> BCM_COM_PROC_P20/158(V_BCM_COM_DBCU_FAILED_Conf_Flt)
  V_BCM_COM_DBCU_FAILED_Unconf_Flt/1 -> BCM_COM_PROC_P20/159(V_BCM_COM_DBCU_FAILED_Unconf_Flt)
  V_BCM_COM_DBCU_ALT_MODE_Conf_Flt/1 -> BCM_COM_PROC_P20/160(V_BCM_COM_DBCU_ALT_MODE_Conf_Flt)
  V_BCM_COM_DBCU_ALT_MODE_Unconf_Flt/1 -> BCM_COM_PROC_P20/161(V_BCM_COM_DBCU_ALT_MODE_Unconf_Flt)
  V_BCM_COM_ACCU_PT_Conf_Flt/1 -> BCM_COM_PROC_P20/162(V_BCM_COM_ACCU_PT_Conf_Flt)
  V_BCM_COM_ACCU_PT_Unconf_Flt/1 -> BCM_COM_PROC_P20/163(V_BCM_COM_ACCU_PT_Unconf_Flt)
  V_BCM_COM_ACCU_PT_Acq/1 -> BCM_COM_PROC_P20/164(V_BCM_COM_ACCU_PT_Acq)
  V_BCM_COM_LH_BTS_TEMP_Comp/1 -> BCM_COM_PROC_P20/228(V_BCM_COM_LH_BTS_TEMP_Comp)
  V_BCM_COM_LH_BTS_Conf_Flt/1 -> BCM_COM_PROC_P20/165(V_BCM_COM_LH_BTS_Conf_Flt)
  V_BCM_COM_LH_BTS_Unconf_Flt/1 -> BCM_COM_PROC_P20/166(V_BCM_COM_LH_BTS_Unconf_Flt)
  V_BCM_COM_RH_BTS_TEMP_Comp/1 -> BCM_COM_PROC_P20/229(V_BCM_COM_RH_BTS_TEMP_Comp)
  V_BCM_COM_RH_BTS_Conf_Flt/1 -> BCM_COM_PROC_P20/167(V_BCM_COM_RH_BTS_Conf_Flt)
  V_BCM_COM_RH_BTS_Unconf_Flt/1 -> BCM_COM_PROC_P20/168(V_BCM_COM_RH_BTS_Unconf_Flt)
  V_BCM_COM_BCP_PARK_OFF_SW_CMD_Acq/1 -> BCM_COM_PROC_P20/169(V_BCM_COM_BCP_PARK_OFF_SW_CMD_Acq)
  V_BCM_COM_BCP_PARK_OFF_SW_CMD_Conf_Flt/1 -> BCM_COM_PROC_P20/170(V_BCM_COM_BCP_PARK_OFF_SW_CMD_Conf_Flt)
  V_BCM_COM_BCP_PARK_OFF_SW_CMD_Unconf_Flt/1 -> BCM_COM_PROC_P20/171(V_BCM_COM_BCP_PARK_OFF_SW_CMD_Unconf_Flt)
  V_BCM_COM_MP_MAINT_MODE_CMD_28V_Acq/1 -> BCM_COM_PROC_P20/172(V_BCM_COM_MP_MAINT_MODE_CMD_28V_Acq)
  V_BCM_COM_MP_MAINT_MODE_CMD_GND_Acq/1 -> BCM_COM_PROC_P20/173(V_BCM_COM_MP_MAINT_MODE_CMD_GND_Acq)
  V_BCM_COM_LNLG_Tire_Press_Acq/1 -> BCM_COM_PROC_P20/174(V_BCM_COM_LNLG_Tire_Press_Acq)
  V_BCM_COM_LNLG_Tire_Press_Conf_Flt/1 -> BCM_COM_PROC_P20/175(V_BCM_COM_LNLG_Tire_Press_Conf_Flt)
  V_BCM_COM_LNLG_Tire_Press_Unconf_Flt/1 -> BCM_COM_PROC_P20/176(V_BCM_COM_LNLG_Tire_Press_Unconf_Flt)
  V_BCM_COM_RNLG_Tire_Press_Acq/1 -> BCM_COM_PROC_P20/177(V_BCM_COM_RNLG_Tire_Press_Acq)
  V_BCM_COM_RNLG_Tire_Press_Conf_Flt/1 -> BCM_COM_PROC_P20/178(V_BCM_COM_RNLG_Tire_Press_Conf_Flt)
  V_BCM_COM_RNLG_Tire_Press_Unconf_Flt/1 -> BCM_COM_PROC_P20/179(V_BCM_COM_RNLG_Tire_Press_Unconf_Flt)
  V_BCM_COM_LMLG_Outboard_Tire_Press_Acq/1 -> BCM_COM_PROC_P20/180(V_BCM_COM_LMLG_Outboard_Tire_Press_Acq)
  V_BCM_COM_LMLG_Outboard_Tire_Press_Conf_Flt/1 -> BCM_COM_PROC_P20/181(V_BCM_COM_LMLG_Outboard_Tire_Press_Conf_Flt)
  V_BCM_COM_LMLG_Outboard_Tire_Press_Unconf_Flt/1 -> BCM_COM_PROC_P20/182(V_BCM_COM_LMLG_Outboard_Tire_Press_Unconf_Flt)
  V_BCM_COM_LMLG_Inboard_Tire_Press_Acq/1 -> BCM_COM_PROC_P20/183(V_BCM_COM_LMLG_Inboard_Tire_Press_Acq)
  V_BCM_COM_LMLG_Inboard_Tire_Press_Conf_Flt/1 -> BCM_COM_PROC_P20/184(V_BCM_COM_LMLG_Inboard_Tire_Press_Conf_Flt)
  V_BCM_COM_LMLG_Inboard_Tire_Press_Unconf_Flt/1 -> BCM_COM_PROC_P20/185(V_BCM_COM_LMLG_Inboard_Tire_Press_Unconf_Flt)
  V_BCM_COM_RMLG_Inboard_Tire_Press_Acq/1 -> BCM_COM_PROC_P20/186(V_BCM_COM_RMLG_Inboard_Tire_Press_Acq)
  V_BCM_COM_RMLG_Inboard_Tire_Press_Conf_Flt/1 -> BCM_COM_PROC_P20/187(V_BCM_COM_RMLG_Inboard_Tire_Press_Conf_Flt)
  V_BCM_COM_RMLG_Inboard_Tire_Press_Unconf_Flt/1 -> BCM_COM_PROC_P20/188(V_BCM_COM_RMLG_Inboard_Tire_Press_Unconf_Flt)
  V_BCM_COM_RMLG_Outboard_Tire_Press_Acq/1 -> BCM_COM_PROC_P20/189(V_BCM_COM_RMLG_Outboard_Tire_Press_Acq)
  V_BCM_COM_RMLG_Outboard_Tire_Press_Conf_Flt/1 -> BCM_COM_PROC_P20/190(V_BCM_COM_RMLG_Outboard_Tire_Press_Conf_Flt)
  V_BCM_COM_RMLG_Outboard_Tire_Press_Unconf_Flt/1 -> BCM_COM_PROC_P20/191(V_BCM_COM_RMLG_Outboard_Tire_Press_Unconf_Flt)
  V_BCM_COM_Whl_AS_Curr_Order/1 -> BCM_COM_PROC_P20/192(V_BCM_COM_Whl_AS_Curr_Order)
  V_BCM_COM_SV_Current_Readback/1 -> BCM_COM_PROC_P20/193(V_BCM_COM_SV_Current_Readback)
  V_BCM_COM_Whl_AS_Activity/1 -> BCM_COM_PROC_P20/194(V_BCM_COM_Whl_AS_Activity)
  V_BCM_COM_SELV_High_Side_Readback_Val/1 -> BCM_COM_PROC_P20/195(V_BCM_COM_SELV_High_Side_Readback_Val)
  V_BCM_COM_SELV_High_Side_Readback/1 -> BCM_COM_PROC_P20/196(V_BCM_COM_SELV_High_Side_Readback)
  V_BCM_COM_CF_LH_SV_SC/1 -> BCM_COM_PROC_P20/197(V_BCM_COM_CF_LH_SV_SC)
  V_BCM_COM_CF_LH_SV_OC/1 -> BCM_COM_PROC_P20/198(V_BCM_COM_CF_LH_SV_OC)
  V_BCM_COM_CF_RH_SV_SC/1 -> BCM_COM_PROC_P20/199(V_BCM_COM_CF_RH_SV_SC)
  V_BCM_COM_CF_RH_SV_OC/1 -> BCM_COM_PROC_P20/200(V_BCM_COM_CF_RH_SV_OC)
  V_BCM_COM_CF_SELV_SC/1 -> BCM_COM_PROC_P20/201(V_BCM_COM_CF_SELV_SC)
  V_BCM_COM_CF_SELV_OC/1 -> BCM_COM_PROC_P20/202(V_BCM_COM_CF_SELV_OC)
  V_BCM_COM_CF_SELV_JOP/1 -> BCM_COM_PROC_P20/203(V_BCM_COM_CF_SELV_JOP)
  V_BCM_COM_CF_SELV_JCL/1 -> BCM_COM_PROC_P20/204(V_BCM_COM_CF_SELV_JCL)
  V_BCM_COM_CF_PARK_BRK/1 -> BCM_COM_PROC_P20/205(V_BCM_COM_CF_PARK_BRK)
  V_BCM_COM_CF_RESIDUAL_PRESS/1 -> BCM_COM_PROC_P20/206(V_BCM_COM_CF_RESIDUAL_PRESS)
  V_BCM_COM_Avionics_Conf_Flt/1 -> BCM_COM_PROC_P20/207(V_BCM_COM_Avionics_Conf_Flt)
  V_BCM_COM_DFCS_A_Conf_Flt/1 -> BCM_COM_PROC_P20/208(V_BCM_COM_DFCS_A_Conf_Flt)
  V_BCM_COM_DFCS_A_DFCS_BCM_Caps_Val/1 -> BCM_COM_PROC_P20/209(V_BCM_COM_DFCS_A_DFCS_BCM_Caps_Val)
  V_BCM_COM_DFCS_B_Conf_Flt/1 -> BCM_COM_PROC_P20/210(V_BCM_COM_DFCS_B_Conf_Flt)
  V_BCM_COM_DFCS_B_DFCS_BCM_Caps_Val/1 -> BCM_COM_PROC_P20/211(V_BCM_COM_DFCS_B_DFCS_BCM_Caps_Val)
  V_BCM_COM_PPRG_i_Acquired/1 -> BCM_COM_PROC_P20/212(V_BCM_COM_PPRG_i_Acquired)
  V_BCM_COM_PPRG_Fault/1 -> BCM_COM_PROC_P20/213(V_BCM_COM_PPRG_Fault)
  V_BCM_COM_DBCU_Conf_Flt/1 -> BCM_COM_PROC_P20/214(V_BCM_COM_DBCU_Conf_Flt)
  V_BCM_COM_SV_Current_Readback_Val/1 -> BCM_COM_PROC_P20/215(V_BCM_COM_SV_Current_Readback_Val)
  V_BCM_COM_SV_Current_Order/1 -> BCM_COM_PROC_P20/216(V_BCM_COM_SV_Current_Order)
  V_BCM_COM_CF_BSELV_OC/1 -> BCM_COM_PROC_P20/217(V_BCM_COM_CF_BSELV_OC)
  V_BCM_COM_CF_BSELV_SC/1 -> BCM_COM_PROC_P20/218(V_BCM_COM_CF_BSELV_SC)
  V_BCM_COM_CF_BSELV_JCL/1 -> BCM_COM_PROC_P20/219(V_BCM_COM_CF_BSELV_JCL)
  V_BCM_COM_CF_BSELV_JOP/1 -> BCM_COM_PROC_P20/220(V_BCM_COM_CF_BSELV_JOP)
  V_BCM_COM_LH_SV_PT_Conf_Flt/1 -> BCM_COM_PROC_P20/221(V_BCM_COM_LH_SV_PT_Conf_Flt)
  V_BCM_COM_CF_SV_DRIFT/1 -> BCM_COM_PROC_P20/222(V_BCM_COM_CF_SV_DRIFT)
  V_BCM_COM_CF_LH_SV_JCL/1 -> BCM_COM_PROC_P20/223(V_BCM_COM_CF_LH_SV_JCL)
  V_BCM_COM_CF_LH_SV_JOP/1 -> BCM_COM_PROC_P20/224(V_BCM_COM_CF_LH_SV_JOP)
  V_BCM_COM_RH_SV_PT_Conf_Flt/1 -> BCM_COM_PROC_P20/225(V_BCM_COM_RH_SV_PT_Conf_Flt)
  V_BCM_COM_CF_RH_SV_JCL/1 -> BCM_COM_PROC_P20/226(V_BCM_COM_CF_RH_SV_JCL)
  V_BCM_COM_CF_RH_SV_JOP/1 -> BCM_COM_PROC_P20/227(V_BCM_COM_CF_RH_SV_JOP)
  BCM_Tuning/1 -> BCM_COM_PROC_P20/230(BCM_Tuning)
  BCM_COM_PROC_P20/1(V_BCM_COM_Whl_Spun_Up_State_W12) -> V_BCM_COM_Whl_Spun_Up_State_W12/1
  BCM_COM_PROC_P20/2(V_BCM_COM_Whl_Ref_Speed_W12) -> V_BCM_COM_Whl_Ref_Speed_W12/1
  BCM_COM_PROC_P20/3(V_BCM_COM_Whl_Spun_Up_State_W34) -> V_BCM_COM_Whl_Spun_Up_State_W34/1
  BCM_COM_PROC_P20/4(V_BCM_COM_Whl_Ref_Speed_W34) -> V_BCM_COM_Whl_Ref_Speed_W34/1
  BCM_COM_PROC_P20/5(V_BCM_COM_DFCS_A_Gnd_Spd_Conv) -> V_BCM_COM_DFCS_A_Gnd_Spd_Conv/1
  BCM_COM_PROC_P20/6(V_BCM_COM_DFCS_B_Gnd_Spd_Conv) -> V_BCM_COM_DFCS_B_Gnd_Spd_Conv/1
  BCM_COM_PROC_P20/7(V_BCM_COM_AC_Gnd_Spd_Cons) -> V_BCM_COM_AC_Gnd_Spd_Cons/1
  BCM_COM_PROC_P20/8(V_BCM_COM_AC_Gnd_Spd_Cons_Val) -> V_BCM_COM_AC_Gnd_Spd_Cons_Val/1
  BCM_COM_PROC_P20/9(V_BCM_COM_DFCS_A_Long_Accel_Conv) -> V_BCM_COM_DFCS_A_Long_Accel_Conv/1
  BCM_COM_PROC_P20/10(V_BCM_COM_DFCS_B_Long_Accel_Conv) -> V_BCM_COM_DFCS_B_Long_Accel_Conv/1
  BCM_COM_PROC_P20/11(V_BCM_COM_AC_Long_Accel_Cons) -> V_BCM_COM_AC_Long_Accel_Cons/1
  BCM_COM_PROC_P20/12(V_BCM_COM_AC_Long_Accel_Cons_Val) -> V_BCM_COM_AC_Long_Accel_Cons_Val/1
  BCM_COM_PROC_P20/13(V_BCM_COM_AC_Long_Accel_Filt_Corr) -> V_BCM_COM_AC_Long_Accel_Filt_Corr/1
  BCM_COM_PROC_P20/14(V_BCM_COM_AC_Pitch_Ang_Cons_Val) -> V_BCM_COM_AC_Pitch_Ang_Cons_Val/1
  BCM_COM_PROC_P20/15(V_BCM_COM_AC_Pitch_Ang_Filt) -> V_BCM_COM_AC_Pitch_Ang_Filt/1
  BCM_COM_PROC_P20/16(V_BCM_COM_AC_Pitch_Ang_Cons) -> V_BCM_COM_AC_Pitch_Ang_Cons/1
  BCM_COM_PROC_P20/17(V_BCM_COM_DFCS_A_WOWs_Val_Cons) -> V_BCM_COM_DFCS_A_WOWs_Val_Cons/1
  BCM_COM_PROC_P20/18(V_BCM_COM_DFCS_B_WOWs_Val_Cons) -> V_BCM_COM_DFCS_B_WOWs_Val_Cons/1
  BCM_COM_PROC_P20/19(V_BCM_COM_LMLG_WOWs_Cons) -> V_BCM_COM_LMLG_WOWs_Cons/1
  BCM_COM_PROC_P20/20(V_BCM_COM_LMLG_WOWs_Cons_Val) -> V_BCM_COM_LMLG_WOWs_Cons_Val/1
  BCM_COM_PROC_P20/21(V_BCM_COM_RMLG_WOWs_Cons) -> V_BCM_COM_RMLG_WOWs_Cons/1
  BCM_COM_PROC_P20/22(V_BCM_COM_RMLG_WOWs_Cons_Val) -> V_BCM_COM_RMLG_WOWs_Cons_Val/1
  BCM_COM_PROC_P20/23(V_BCM_COM_NLG_WOWs_Cons) -> V_BCM_COM_NLG_WOWs_Cons/1
  BCM_COM_PROC_P20/24(V_BCM_COM_NLG_WOWs_Cons_Val) -> V_BCM_COM_NLG_WOWs_Cons_Val/1
  BCM_COM_PROC_P20/25(V_BCM_COM_LMLG_On_Gnd_State) -> V_BCM_COM_LMLG_On_Gnd_State/1
  BCM_COM_PROC_P20/26(V_BCM_COM_RMLG_On_Gnd_State) -> V_BCM_COM_RMLG_On_Gnd_State/1
  BCM_COM_PROC_P20/27(V_BCM_COM_LMLG_On_Gnd_State_Val) -> V_BCM_COM_LMLG_On_Gnd_State_Val/1
  BCM_COM_PROC_P20/28(V_BCM_COM_RMLG_On_Gnd_State_Val) -> V_BCM_COM_RMLG_On_Gnd_State_Val/1
  BCM_COM_PROC_P20/29(V_BCM_COM_MLG_On_Gnd_State) -> V_BCM_COM_MLG_On_Gnd_State/1
  BCM_COM_PROC_P20/30(V_BCM_COM_NLG_On_Gnd_State) -> V_BCM_COM_NLG_On_Gnd_State/1
  BCM_COM_PROC_P20/31(V_BCM_COM_NLG_On_Gnd_State_Val) -> V_BCM_COM_NLG_On_Gnd_State_Val/1
  BCM_COM_PROC_P20/32(V_BCM_COM_NLG_On_Gnd_State_Cons) -> V_BCM_COM_NLG_On_Gnd_State_Cons/1
  BCM_COM_PROC_P20/33(V_BCM_COM_LH_Braking_Cmd_Cons) -> V_BCM_COM_LH_Braking_Cmd_Cons/1
  BCM_COM_PROC_P20/34(V_BCM_COM_RH_Braking_Cmd_Cons) -> V_BCM_COM_RH_Braking_Cmd_Cons/1
  BCM_COM_PROC_P20/35(V_BCM_COM_Decel_Law_Inhib_Cons) -> V_BCM_COM_Decel_Law_Inhib_Cons/1
  BCM_COM_PROC_P20/36(V_BCM_COM_Decel_Law_Inhib_Cons_Val) -> V_BCM_COM_Decel_Law_Inhib_Cons_Val/1
  BCM_COM_PROC_P20/37(V_BCM_COM_TLA_State_Cons) -> V_BCM_COM_TLA_State_Cons/1
  BCM_COM_PROC_P20/38(V_BCM_COM_TLA_State_Cons_Val) -> V_BCM_COM_TLA_State_Cons_Val/1
  BCM_COM_PROC_P20/39(V_BCM_COM_LG_Lever_Up_Conf) -> V_BCM_COM_LG_Lever_Up_Conf/1
  BCM_COM_PROC_P20/40(V_BCM_COM_LG_Lever_State_Cons) -> V_BCM_COM_LG_Lever_State_Cons/1
  BCM_COM_PROC_P20/41(V_BCM_COM_LG_Lever_Ste_Cons_Val) -> V_BCM_COM_LG_Lever_Ste_Cons_Val/1
  BCM_COM_PROC_P20/42(V_BCM_COM_LMLG_Downlock_Conf) -> V_BCM_COM_LMLG_Downlock_Conf/1
  BCM_COM_PROC_P20/43(V_BCM_COM_RMLG_Downlock_Conf) -> V_BCM_COM_RMLG_Downlock_Conf/1
  BCM_COM_PROC_P20/44(V_BCM_COM_LMLG_Downlock_State) -> V_BCM_COM_LMLG_Downlock_State/1
  BCM_COM_PROC_P20/45(V_BCM_COM_LMLG_Dnlk_State_Val) -> V_BCM_COM_LMLG_Dnlk_State_Val/1
  BCM_COM_PROC_P20/46(V_BCM_COM_RMLG_Downlock_State) -> V_BCM_COM_RMLG_Downlock_State/1
  BCM_COM_PROC_P20/47(V_BCM_COM_RMLG_Dnlk_State_Val) -> V_BCM_COM_RMLG_Dnlk_State_Val/1
  BCM_COM_PROC_P20/48(V_BCM_COM_SELV_High_Side_Cmd_Order) -> V_BCM_COM_SELV_High_Side_Cmd_Order/1
  BCM_COM_PROC_P20/49(V_BCM_COM_SELV_Low_Speed_Logic) -> V_BCM_COM_SELV_Low_Speed_Logic/1
  BCM_COM_PROC_P20/50(V_BCM_COM_Engine_State) -> V_BCM_COM_Engine_State/1
  BCM_COM_PROC_P20/51(V_BCM_COM_Engine_State_Val) -> V_BCM_COM_Engine_State_Val/1
  BCM_COM_PROC_P20/52(V_BCM_COM_LH_Braking_Cmd_State) -> V_BCM_COM_LH_Braking_Cmd_State/1
  BCM_COM_PROC_P20/53(V_BCM_COM_RH_Braking_Cmd_State) -> V_BCM_COM_RH_Braking_Cmd_State/1
  BCM_COM_PROC_P20/54(V_BCM_COM_LH_Regular_Brkg_Press_Cmd) -> V_BCM_COM_LH_Regular_Brkg_Press_Cmd/1
  BCM_COM_PROC_P20/55(V_BCM_COM_RH_Regular_Brkg_Press_Cmd) -> V_BCM_COM_RH_Regular_Brkg_Press_Cmd/1
  BCM_COM_PROC_P20/56(V_BCM_COM_Wheels_Global_Spun_Up_Ste) -> V_BCM_COM_Wheels_Global_Spun_Up_Ste/1
  BCM_COM_PROC_P20/57(V_BCM_COM_Global_Reference_Spd) -> V_BCM_COM_Global_Reference_Spd/1
  BCM_COM_PROC_P20/58(V_BCM_COM_Global_Wheel_Spd) -> V_BCM_COM_Global_Wheel_Spd/1
  BCM_COM_PROC_P20/59(V_BCM_COM_LMLG_Global_Wheel_Spd) -> V_BCM_COM_LMLG_Global_Wheel_Spd/1
  BCM_COM_PROC_P20/60(V_BCM_COM_RMLG_Global_Wheel_Spd) -> V_BCM_COM_RMLG_Global_Wheel_Spd/1
  BCM_COM_PROC_P20/61(V_BCM_COM_AC_State) -> V_BCM_COM_AC_State/1
  BCM_COM_PROC_P20/62(V_BCM_COM_AC_Flight_Phase) -> V_BCM_COM_AC_Flight_Phase/1
  BCM_COM_PROC_P20/63(V_BCM_COM_Braking_Mode) -> V_BCM_COM_Braking_Mode/1
  BCM_COM_PROC_P20/64(v_BCM_COM_FT_Seq) -> v_BCM_COM_FT_Seq/1
  BCM_COM_PROC_P20/65(V_BCM_COM_Start_Norm_FT_Cond) -> V_BCM_COM_Start_Norm_FT_Cond/1
  BCM_COM_PROC_P20/66(V_BCM_COM_Brkg_Norm_FT_Prog_Sts) -> V_BCM_COM_Brkg_Norm_FT_Prog_Sts/1
  BCM_COM_PROC_P20/67(V_BCM_COM_Brkg_Norm_FT_Cond) -> V_BCM_COM_Brkg_Norm_FT_Cond/1
  BCM_COM_PROC_P20/68(V_BCM_COM_Braking_Norm_FT_Seq) -> V_BCM_COM_Braking_Norm_FT_Seq/1
  BCM_COM_PROC_P20/69(V_BCM_COM_Abort_Norm_FT_Cond) -> V_BCM_COM_Abort_Norm_FT_Cond/1
  BCM_COM_PROC_P20/70(V_BCM_COM_Brkg_Alt_FT_Prog_Sts) -> V_BCM_COM_Brkg_Alt_FT_Prog_Sts/1
  BCM_COM_PROC_P20/71(V_BCM_COM_Braking_Alt_FT_Seq) -> V_BCM_COM_Braking_Alt_FT_Seq/1
  BCM_COM_PROC_P20/72(V_BCM_COM_Abort_Alt_FT_Cond) -> V_BCM_COM_Abort_Alt_FT_Cond/1
  BCM_COM_PROC_P20/73(V_BCM_COM_Start_Alt_FT_Cond) -> V_BCM_COM_Start_Alt_FT_Cond/1
  BCM_COM_PROC_P20/74(V_BCM_COM_Brkg_Alt_FT_Cond) -> V_BCM_COM_Brkg_Alt_FT_Cond/1
  BCM_COM_PROC_P20/75(V_BCM_COM_LH_Press_Reg_FT_Act_Cond) -> V_BCM_COM_LH_Press_Reg_FT_Act_Cond/1
  BCM_COM_PROC_P20/76(V_BCM_COM_RH_Press_Reg_FT_Act_Cond) -> V_BCM_COM_RH_Press_Reg_FT_Act_Cond/1
  BCM_COM_PROC_P20/77(V_BCM_COM_LH_Press_Law_Brkg_Press_Cmd) -> V_BCM_COM_LH_Press_Law_Brkg_Press_Cmd/1
  BCM_COM_PROC_P20/78(V_BCM_COM_RH_Press_Law_Brkg_Press_Cmd) -> V_BCM_COM_RH_Press_Law_Brkg_Press_Cmd/1
  BCM_COM_PROC_P20/79(V_BCM_COM_LH_FT_Press_Cmd) -> V_BCM_COM_LH_FT_Press_Cmd/1
  BCM_COM_PROC_P20/80(V_BCM_COM_RH_FT_Press_Cmd) -> V_BCM_COM_RH_FT_Press_Cmd/1
  BCM_COM_PROC_P20/81(V_BCM_COM_LH_Ret_Brkg_Press_Cmd) -> V_BCM_COM_LH_Ret_Brkg_Press_Cmd/1
  BCM_COM_PROC_P20/82(V_BCM_COM_RH_Ret_Brkg_Press_Cmd) -> V_BCM_COM_RH_Ret_Brkg_Press_Cmd/1
  BCM_COM_PROC_P20/83(V_BCM_COM_LH_Eng_Run_Press_Cmd) -> V_BCM_COM_LH_Eng_Run_Press_Cmd/1
  BCM_COM_PROC_P20/84(V_BCM_COM_RH_Eng_Run_Press_Cmd) -> V_BCM_COM_RH_Eng_Run_Press_Cmd/1
  BCM_COM_PROC_P20/85(V_BCM_COM_Brkg_SELV_High_Side_FT_Cmd_Order) -> V_BCM_COM_Brkg_SELV_High_Side_FT_Cmd_Order/1
  BCM_COM_PROC_P20/86(V_BCM_COM_DBCU_FT_Inhib_Order) -> V_BCM_COM_DBCU_FT_Inhib_Order/1
  BCM_COM_PROC_P20/87(V_BCM_COM_DBCU_Inhib_Order) -> V_BCM_COM_DBCU_Inhib_Order/1
  BCM_COM_PROC_P20/88(V_BCM_COM_BCM_Validity) -> V_BCM_COM_BCM_Validity/1
  BCM_COM_PROC_P20/89(V_BCM_COM_Alt_Sw_Cmd_Cons) -> V_BCM_COM_Alt_Sw_Cmd_Cons/1
  BCM_COM_PROC_P20/90(V_BCM_COM_Alt_Sw_Cmd_Cons_Val) -> V_BCM_COM_Alt_Sw_Cmd_Cons_Val/1
  BCM_COM_PROC_P20/91(V_BCM_COM_Disp_Sw_Cmd_Cons) -> V_BCM_COM_Disp_Sw_Cmd_Cons/1
  BCM_COM_PROC_P20/92(V_BCM_COM_Disp_Sw_Cmd_Cons_Val) -> V_BCM_COM_Disp_Sw_Cmd_Cons_Val/1
  BCM_COM_PROC_P20/93(V_BCM_COM_MP_BCMA_Alt_Disp_Sw_Conf) -> V_BCM_COM_MP_BCMA_Alt_Disp_Sw_Conf/1
  BCM_COM_PROC_P20/94(V_BCM_COM_BCP_BCM_Alt_Sw_On_Cmd_Conf) -> V_BCM_COM_BCP_BCM_Alt_Sw_On_Cmd_Conf/1
  BCM_COM_PROC_P20/95(V_BCM_COM_Braking_State) -> V_BCM_COM_Braking_State/1
  BCM_COM_PROC_P20/96(V_BCM_COM_Norm_Brkg_Availability) -> V_BCM_COM_Norm_Brkg_Availability/1
  BCM_COM_PROC_P20/97(V_BCM_COM_Alt_Brkg_Availability) -> V_BCM_COM_Alt_Brkg_Availability/1
  BCM_COM_PROC_P20/98(V_BCM_COM_Braking_Type) -> V_BCM_COM_Braking_Type/1
  BCM_COM_PROC_P20/99(V_BCM_COM_Press_Cmd) -> V_BCM_COM_Press_Cmd/1
  BCM_COM_PROC_P20/100(V_BCM_COM_Brkg_On_Wheels) -> V_BCM_COM_Brkg_On_Wheels/1
  BCM_COM_PROC_P20/101(V_BCM_COM_Press_Cmd_Rate_Lim) -> V_BCM_COM_Press_Cmd_Rate_Lim/1
  BCM_COM_PROC_P20/102(V_BCM_COM_PBSELV_ON_POS_Conf) -> V_BCM_COM_PBSELV_ON_POS_Conf/1
  BCM_COM_PROC_P20/103(V_BCM_COM_PBSELV_State_Cons) -> V_BCM_COM_PBSELV_State_Cons/1
  BCM_COM_PROC_P20/104(V_BCM_COM_PBSELV_State_Cons_Val) -> V_BCM_COM_PBSELV_State_Cons_Val/1
  BCM_COM_PROC_P20/105(V_BCM_COM_Hyd_A_Press_Cons) -> V_BCM_COM_Hyd_A_Press_Cons/1
  BCM_COM_PROC_P20/106(V_BCM_COM_Hyd_B_Press_Cons) -> V_BCM_COM_Hyd_B_Press_Cons/1
  BCM_COM_PROC_P20/107(V_BCM_COM_Hyd_A_Press_Cons_Val) -> V_BCM_COM_Hyd_A_Press_Cons_Val/1
  BCM_COM_PROC_P20/108(V_BCM_COM_Hyd_B_Press_Cons_Val) -> V_BCM_COM_Hyd_B_Press_Cons_Val/1
  BCM_COM_PROC_P20/109(V_BCM_COM_Hyd_A_Press_State) -> V_BCM_COM_Hyd_A_Press_State/1
  BCM_COM_PROC_P20/110(V_BCM_COM_Hyd_B_Press_State) -> V_BCM_COM_Hyd_B_Press_State/1
  BCM_COM_PROC_P20/111(V_BCM_COM_Sys_Sanc_Inhib_During_FT) -> V_BCM_COM_Sys_Sanc_Inhib_During_FT/1
  BCM_COM_PROC_P20/112(V_BCM_COM_Wheel_Control_Speed_W12) -> V_BCM_COM_Wheel_Control_Speed_W12/1
  BCM_COM_PROC_P20/113(V_BCM_COM_Wheel_Control_Speed_W34) -> V_BCM_COM_Wheel_Control_Speed_W34/1
  BCM_COM_PROC_P20/114(V_BCM_COM_Big_Gamma_Trig_Out_W12) -> V_BCM_COM_Big_Gamma_Trig_Out_W12/1
  BCM_COM_PROC_P20/115(V_BCM_COM_Big_Gamma_Trig_Out_W34) -> V_BCM_COM_Big_Gamma_Trig_Out_W34/1
  BCM_COM_PROC_P20/116(V_BCM_COM_Big_Slip_Trig_Out_W12) -> V_BCM_COM_Big_Slip_Trig_Out_W12/1
  BCM_COM_PROC_P20/117(V_BCM_COM_Big_Slip_Trig_Out_W34) -> V_BCM_COM_Big_Slip_Trig_Out_W34/1
  BCM_COM_PROC_P20/118(V_BCM_COM_Big_Slip_WD_Trig_Out_W12) -> V_BCM_COM_Big_Slip_WD_Trig_Out_W12/1
  BCM_COM_PROC_P20/119(V_BCM_COM_Big_Slip_WD_Trig_Out_W34) -> V_BCM_COM_Big_Slip_WD_Trig_Out_W34/1
  BCM_COM_PROC_P20/120(V_BCM_COM_Small_Slip_Trig_Out_W12) -> V_BCM_COM_Small_Slip_Trig_Out_W12/1
  BCM_COM_PROC_P20/121(V_BCM_COM_Small_Slip_Trig_Out_W34) -> V_BCM_COM_Small_Slip_Trig_Out_W34/1
  BCM_COM_PROC_P20/122(V_BCM_COM_Automate_State_W12) -> V_BCM_COM_Automate_State_W12/1
  BCM_COM_PROC_P20/123(V_BCM_COM_Automate_State_W34) -> V_BCM_COM_Automate_State_W34/1
  BCM_COM_PROC_P20/124(V_BCM_COM_Target_Speed_Out_W12) -> V_BCM_COM_Target_Speed_Out_W12/1
  BCM_COM_PROC_P20/125(V_BCM_COM_Target_Speed_Out_W34) -> V_BCM_COM_Target_Speed_Out_W34/1
  BCM_COM_PROC_P20/126(V_BCM_COM_Target_Decel_Out_W12) -> V_BCM_COM_Target_Decel_Out_W12/1
  BCM_COM_PROC_P20/127(V_BCM_COM_Target_Decel_Out_W34) -> V_BCM_COM_Target_Decel_Out_W34/1
  BCM_COM_PROC_P20/128(V_BCM_COM_Adhesion_Out_W12) -> V_BCM_COM_Adhesion_Out_W12/1
  BCM_COM_PROC_P20/129(V_BCM_COM_Adhesion_Out_W34) -> V_BCM_COM_Adhesion_Out_W34/1
  BCM_COM_PROC_P20/130(V_BCM_COM_Opt_Adhesion_Out_W12) -> V_BCM_COM_Opt_Adhesion_Out_W12/1
  BCM_COM_PROC_P20/131(V_BCM_COM_Opt_Adhesion_Out_W34) -> V_BCM_COM_Opt_Adhesion_Out_W34/1
  BCM_COM_PROC_P20/132(V_BCM_COM_Whl_AS_Adp_Gain_W12) -> V_BCM_COM_Whl_AS_Adp_Gain_W12/1
  BCM_COM_PROC_P20/133(V_BCM_COM_Whl_AS_Adp_Gain_W34) -> V_BCM_COM_Whl_AS_Adp_Gain_W34/1
  BCM_COM_PROC_P20/134(V_BCM_COM_Adhesion_In_Cons_W12) -> V_BCM_COM_Adhesion_In_Cons_W12/1
  BCM_COM_PROC_P20/135(V_BCM_COM_Adhesion_In_Cons_W34) -> V_BCM_COM_Adhesion_In_Cons_W34/1
  BCM_COM_PROC_P20/136(V_BCM_COM_Opt_Adhesion_In_Cons_W12) -> V_BCM_COM_Opt_Adhesion_In_Cons_W12/1
  BCM_COM_PROC_P20/137(V_BCM_COM_Opt_Adhesion_In_Cons_W34) -> V_BCM_COM_Opt_Adhesion_In_Cons_W34/1
  BCM_COM_PROC_P20/138(V_BCM_COM_Target_Speed_In_Cons_W12) -> V_BCM_COM_Target_Speed_In_Cons_W12/1
  BCM_COM_PROC_P20/139(V_BCM_COM_Target_Speed_In_Cons_W34) -> V_BCM_COM_Target_Speed_In_Cons_W34/1
  BCM_COM_PROC_P20/140(V_BCM_COM_Big_Slip_WD_Trig_In_Cons_W12) -> V_BCM_COM_Big_Slip_WD_Trig_In_Cons_W12/1
  BCM_COM_PROC_P20/141(V_BCM_COM_Big_Slip_WD_Trig_In_Cons_W34) -> V_BCM_COM_Big_Slip_WD_Trig_In_Cons_W34/1
  BCM_COM_PROC_P20/142(V_BCM_COM_Big_Gamma_Trig_In_Cons_W12) -> V_BCM_COM_Big_Gamma_Trig_In_Cons_W12/1
  BCM_COM_PROC_P20/143(V_BCM_COM_Big_Gamma_Trig_In_Cons_W34) -> V_BCM_COM_Big_Gamma_Trig_In_Cons_W34/1
  BCM_COM_PROC_P20/144(V_BCM_COM_Small_Slip_Trig_In_Cons_W12) -> V_BCM_COM_Small_Slip_Trig_In_Cons_W12/1
  BCM_COM_PROC_P20/145(V_BCM_COM_Small_Slip_Trig_In_Cons_W34) -> V_BCM_COM_Small_Slip_Trig_In_Cons_W34/1
  BCM_COM_PROC_P20/146(V_BCM_COM_Big_Slip_Trig_In_Cons_W12) -> V_BCM_COM_Big_Slip_Trig_In_Cons_W12/1
  BCM_COM_PROC_P20/147(V_BCM_COM_Big_Slip_Trig_In_Cons_W34) -> V_BCM_COM_Big_Slip_Trig_In_Cons_W34/1
  BCM_COM_PROC_P20/148(V_BCM_COM_CCDL_Data_From_Opp_BCM_Val) -> V_BCM_COM_CCDL_Data_From_Opp_BCM_Val/1
  BCM_COM_PROC_P20/149(V_BCM_COM_DBCU_Inhibition_Order_From_Opp_BCM_Cons) -> V_BCM_COM_DBCU_Inhibition_Order_From_Opp_BCM_Cons/1
  BCM_COM_PROC_P20/150(V_BCM_COM_DBCU_Inhibition_Order_From_Opp_BCM_Cons_Val) -> V_BCM_COM_DBCU_Inhibition_Order_From_Opp_BCM_Cons_Val/1
  BCM_COM_PROC_P20/151(V_BCM_COM_Engine_Running_Conf_Flt) -> V_BCM_COM_Engine_Running_Conf_Flt/1
  BCM_COM_PROC_P20/152(V_BCM_COM_Engine_Running_Unconf_Flt) -> V_BCM_COM_Engine_Running_Unconf_Flt/1
  BCM_COM_PROC_P20/153(V_BCM_COM_Hyd_A_Press_Conf_Flt) -> V_BCM_COM_Hyd_A_Press_Conf_Flt/1
  BCM_COM_PROC_P20/154(V_BCM_COM_Hyd_B_Press_Conf_Flt) -> V_BCM_COM_Hyd_B_Press_Conf_Flt/1
  BCM_COM_PROC_P20/155(V_BCM_COM_Hyd_A_Press_Unconf_Flt) -> V_BCM_COM_Hyd_A_Press_Unconf_Flt/1
  BCM_COM_PROC_P20/156(V_BCM_COM_Hyd_B_Press_Unconf_Flt) -> V_BCM_COM_Hyd_B_Press_Unconf_Flt/1
  BCM_COM_PROC_P20/157(V_BCM_COM_DFCS_A_AC_Gnd_Spd_Val) -> V_BCM_COM_DFCS_A_AC_Gnd_Spd_Val/1
  BCM_COM_PROC_P20/158(V_BCM_COM_DFCS_A_AC_Long_Accel_Val) -> V_BCM_COM_DFCS_A_AC_Long_Accel_Val1/1
  BCM_COM_PROC_P20/159(V_BCM_COM_DFCS_A_AC_Pitch_Angle_Val) -> V_BCM_COM_DFCS_A_AC_Pitch_Angle_Val1/1
  BCM_COM_PROC_P20/160(V_BCM_COM_DFCS_A_Decel_Law_Inhib_Val) -> V_BCM_COM_DFCS_A_Decel_Law_Inhib_Val1/1
  BCM_COM_PROC_P20/161(V_BCM_COM_DFCS_B_Decel_Law_Inhib_Val) -> V_BCM_COM_DFCS_B_Decel_Law_Inhib_Val1/1
  BCM_COM_PROC_P20/162(V_BCM_COM_DFCS_B_AC_Gnd_Spd_Val) -> V_BCM_COM_DFCS_B_AC_Gnd_Spd_Val/1
  BCM_COM_PROC_P20/163(V_BCM_COM_DFCS_B_AC_Long_Accel_Val) -> V_BCM_COM_DFCS_B_AC_Long_Accel_Val1/1
  BCM_COM_PROC_P20/164(V_BCM_COM_DFCS_B_AC_Pitch_Angle_Val) -> V_BCM_COM_DFCS_B_AC_Pitch_Angle_Val1/1
  BCM_COM_PROC_P20/165(V_BCM_COM_DFCS_A_LMLG_WOWs_Val) -> V_BCM_COM_DFCS_A_LMLG_WOWs_Val1/1
  BCM_COM_PROC_P20/166(V_BCM_COM_DFCS_A_RMLG_WOWs_Val) -> V_BCM_COM_DFCS_A_RMLG_WOWs_Val1/1
  BCM_COM_PROC_P20/167(V_BCM_COM_DFCS_A_NLG_WOWs_Val) -> V_BCM_COM_DFCS_A_NLG_WOWs_Val1/1
  BCM_COM_PROC_P20/168(V_BCM_COM_DFCS_A_WOWs_Val_Val) -> V_BCM_COM_DFCS_A_WOWs_Val_Val1/1
  BCM_COM_PROC_P20/169(V_BCM_COM_DFCS_B_LMLG_WOWs_Val) -> V_BCM_COM_DFCS_B_LMLG_WOWs_Val1/1
  BCM_COM_PROC_P20/170(V_BCM_COM_DFCS_B_RMLG_WOWs_Val) -> V_BCM_COM_DFCS_B_RMLG_WOWs_Val1/1
  BCM_COM_PROC_P20/171(V_BCM_COM_DFCS_B_NLG_WOWs_Val) -> V_BCM_COM_DFCS_B_NLG_WOWs_Val1/1
  BCM_COM_PROC_P20/172(V_BCM_COM_DFCS_B_WOWs_Val_Val) -> V_BCM_COM_DFCS_B_WOWs_Val_Val1/1
  BCM_COM_PROC_P20/173(V_BCM_COM_DFCS_A_LH_Braking_Cmd_Val) -> V_BCM_COM_DFCS_A_LH_Braking_Cmd_Val1/1
  BCM_COM_PROC_P20/174(V_BCM_COM_DFCS_A_RH_Braking_Cmd_Val) -> V_BCM_COM_DFCS_A_RH_Braking_Cmd_Val1/1
  BCM_COM_PROC_P20/175(V_BCM_COM_DFCS_B_LH_Braking_Cmd_Val) -> V_BCM_COM_DFCS_B_LH_Braking_Cmd_Val1/1
  BCM_COM_PROC_P20/176(V_BCM_COM_DFCS_B_RH_Braking_Cmd_Val) -> V_BCM_COM_DFCS_B_RH_Braking_Cmd_Val1/1
  BCM_COM_PROC_P20/177(V_BCM_COM_DFCS_A_DBCU_Alt_Mode_1_Val) -> V_BCM_COM_DFCS_A_DBCU_Alt_Mode_1_Val/1
  BCM_COM_PROC_P20/178(V_BCM_COM_DFCS_A_DBCU_Alt_Mode_2_Val) -> V_BCM_COM_DFCS_A_DBCU_Alt_Mode_2_Val/1
  BCM_COM_PROC_P20/179(V_BCM_COM_DFCS_B_DBCU_Alt_Mode_1_Val) -> V_BCM_COM_DFCS_B_DBCU_Alt_Mode_1_Val/1
  BCM_COM_PROC_P20/180(V_BCM_COM_DFCS_B_DBCU_Alt_Mode_2_Val) -> V_BCM_COM_DFCS_B_DBCU_Alt_Mode_2_Val/1
  BCM_COM_PROC_P20/181(V_BCM_COM_DFCS_A_TLA_Above_Idle_Val) -> V_BCM_COM_DFCS_A_TLA_Above_Idle_Val1/1
  BCM_COM_PROC_P20/182(V_BCM_COM_DFCS_B_TLA_Above_Idle_Val) -> V_BCM_COM_DFCS_B_TLA_Above_Idle_Val1/1
  BCM_COM_PROC_P20/183(V_BCM_COM_UTC_Time_Hours_Cons) -> V_BCM_COM_UTC_Time_Hours_Cons/1
  BCM_COM_PROC_P20/184(V_BCM_COM_UTC_Time_Hours_Cons_Val) -> V_BCM_COM_UTC_Time_Hours_Cons_Val/1
  BCM_COM_PROC_P20/185(V_BCM_COM_UTC_Time_Minutes_Cons) -> V_BCM_COM_UTC_Time_Minutes_Cons/1
  BCM_COM_PROC_P20/186(V_BCM_COM_UTC_Time_Minutes_Cons_Val) -> V_BCM_COM_UTC_Time_Minutes_Cons_Val/1
  BCM_COM_PROC_P20/187(V_BCM_COM_UTC_Time_Seconds_Cons) -> V_BCM_COM_UTC_Time_Seconds_Cons/1
  BCM_COM_PROC_P20/188(V_BCM_COM_UTC_Time_Seconds_Cons_Val) -> V_BCM_COM_UTC_Time_Seconds_Cons_Val/1
  BCM_COM_PROC_P20/189(V_BCM_COM_DBCU_BRK_ORDER_FAIL_Conf) -> V_BCM_COM_DBCU_BRK_ORDER_FAIL_Conf/1
  BCM_COM_PROC_P20/190(V_BCM_COM_DBCU_DISPATCH_SW_ON_Conf) -> V_BCM_COM_DBCU_DISPATCH_SW_ON_Conf/1
  BCM_COM_PROC_P20/191(V_BCM_COM_LH_DBCU_BRK_CMD_FDBK_Conf) -> V_BCM_COM_LH_DBCU_BRK_CMD_FDBK_Conf/1
  BCM_COM_PROC_P20/192(V_BCM_COM_RH_DBCU_BRK_CMD_FDBK_Conf) -> V_BCM_COM_RH_DBCU_BRK_CMD_FDBK_Conf/1
  BCM_COM_PROC_P20/193(V_BCM_COM_DBCU_FAILED_Conf) -> V_BCM_COM_DBCU_FAILED_Conf/1
  BCM_COM_PROC_P20/194(V_BCM_COM_DBCU_ALT_MODE_Conf) -> V_BCM_COM_DBCU_ALT_MODE_Conf/1
  BCM_COM_PROC_P20/195(V_BCM_COM_DBCU_BRK_ORDER_FAIL_Cons) -> V_BCM_COM_DBCU_BRK_ORDER_FAIL_Cons/1
  BCM_COM_PROC_P20/196(V_BCM_COM_DBCU_BRK_ORDER_FAIL_Cons_Val) -> V_BCM_COM_DBCU_BRK_ORDER_FAIL_Cons_Val/1
  BCM_COM_PROC_P20/197(V_BCM_COM_DBCU_DISPATCH_SW_ON_Cons) -> V_BCM_COM_DBCU_DISPATCH_SW_ON_Cons/1
  BCM_COM_PROC_P20/198(V_BCM_COM_DBCU_DISPATCH_SW_ON_Cons_Val) -> V_BCM_COM_DBCU_DISPATCH_SW_ON_Cons_Val/1
  BCM_COM_PROC_P20/199(V_BCM_COM_LH_DBCU_BRK_CMD_FDBK_Cons) -> V_BCM_COM_LH_DBCU_BRK_CMD_FDBK_Cons/1
  BCM_COM_PROC_P20/200(V_BCM_COM_LH_DBCU_BRK_CMD_FDBK_Cons_Val) -> V_BCM_COM_LH_DBCU_BRK_CMD_FDBK_Cons_Val/1
  BCM_COM_PROC_P20/201(V_BCM_COM_RH_DBCU_BRK_CMD_FDBK_Cons) -> V_BCM_COM_RH_DBCU_BRK_CMD_FDBK_Cons/1
  BCM_COM_PROC_P20/202(V_BCM_COM_RH_DBCU_BRK_CMD_FDBK_Cons_Val) -> V_BCM_COM_RH_DBCU_BRK_CMD_FDBK_Cons_Val/1
  BCM_COM_PROC_P20/203(V_BCM_COM_DBCU_FAILED_Cons) -> V_BCM_COM_DBCU_FAILED_Cons/1
  BCM_COM_PROC_P20/204(V_BCM_COM_DBCU_FAILED_Cons_Val) -> V_BCM_COM_DBCU_FAILED_Cons_Val/1
  BCM_COM_PROC_P20/205(V_BCM_COM_DBCU_ALT_MODE_Cons) -> V_BCM_COM_DBCU_ALT_MODE_Cons/1
  BCM_COM_PROC_P20/206(V_BCM_COM_DBCU_ALT_MODE_Cons_Val) -> V_BCM_COM_DBCU_ALT_MODE_Cons_Val/1
  BCM_COM_PROC_P20/207(V_BCM_COM_ACCU_PT_Cons) -> V_BCM_COM_ACCU_PT_Cons/1
  BCM_COM_PROC_P20/208(V_BCM_COM_ACCU_PT_Cons_Val) -> V_BCM_COM_ACCU_PT_Cons_Val/1
  BCM_COM_PROC_P20/209(V_BCM_COM_ACCU_Pressure_State) -> V_BCM_COM_ACCU_Pressure_State/1
  BCM_COM_PROC_P20/210(V_BCM_COM_LH_Brake_Temp_Cons) -> V_BCM_COM_LH_Brake_Temp_Cons/1
  BCM_COM_PROC_P20/211(V_BCM_COM_LH_Brake_Temp_Cons_Val) -> V_BCM_COM_LH_Brake_Temp_Cons_Val/1
  BCM_COM_PROC_P20/212(V_BCM_COM_RH_Brake_Temp_Cons) -> V_BCM_COM_RH_Brake_Temp_Cons/1
  BCM_COM_PROC_P20/213(V_BCM_COM_RH_Brake_Temp_Cons_Val) -> V_BCM_COM_RH_Brake_Temp_Cons_Val/1
  BCM_COM_PROC_P20/214(V_BCM_COM_BCP_PARK_OFF_SW_CMD_Conf) -> V_BCM_COM_BCP_PARK_OFF_SW_CMD_Conf/1
  BCM_COM_PROC_P20/215(V_BCM_COM_Park_Sw_Cmd_Cons) -> V_BCM_COM_Park_Sw_Cmd_Cons/1
  BCM_COM_PROC_P20/216(V_BCM_COM_Park_Sw_Cmd_Cons_Val) -> V_BCM_COM_Park_Sw_Cmd_Cons_Val/1
  BCM_COM_PROC_P20/217(V_BCM_COM_MP_MAINT_MODE_CMD_28V_Conf) -> V_BCM_COM_MP_MAINT_MODE_CMD_28V_Conf/1
  BCM_COM_PROC_P20/218(V_BCM_COM_MP_MAINT_MODE_CMD_GND_Conf) -> V_BCM_COM_MP_MAINT_MODE_CMD_GND_Conf/1
  BCM_COM_PROC_P20/219(V_BCM_COM_Maint_Mode_State_Cons) -> V_BCM_COM_Maint_Mode_State_Cons/1
  BCM_COM_PROC_P20/220(V_BCM_COM_LNLG_Tire_Press_Cons) -> V_BCM_COM_LNLG_Tire_Press_Cons/1
  BCM_COM_PROC_P20/221(V_BCM_COM_RNLG_Tire_Press_Cons) -> V_BCM_COM_RNLG_Tire_Press_Cons/1
  BCM_COM_PROC_P20/222(V_BCM_COM_LNLG_Tire_Press_Cons_Val) -> V_BCM_COM_LNLG_Tire_Press_Cons_Val/1
  BCM_COM_PROC_P20/223(V_BCM_COM_RNLG_Tire_Press_Cons_Val) -> V_BCM_COM_RNLG_Tire_Press_Cons_Val/1
  BCM_COM_PROC_P20/224(V_BCM_COM_LMLG_Outboard_Tire_Press_Cons) -> V_BCM_COM_LMLG_Outboard_Tire_Press_Cons/1
  BCM_COM_PROC_P20/225(V_BCM_COM_LMLG_Outboard_Tire_Press_Cons_Val) -> V_BCM_COM_LMLG_Outboard_Tire_Press_Cons_Val/1
  BCM_COM_PROC_P20/226(V_BCM_COM_LMLG_Inboard_Tire_Press_Cons) -> V_BCM_COM_LMLG_Inboard_Tire_Press_Cons/1
  BCM_COM_PROC_P20/227(V_BCM_COM_LMLG_Inboard_Tire_Press_Cons_Val) -> V_BCM_COM_LMLG_Inboard_Tire_Press_Cons_Val/1
  BCM_COM_PROC_P20/228(V_BCM_COM_RMLG_Inboard_Tire_Press_Cons) -> V_BCM_COM_RMLG_Inboard_Tire_Press_Cons/1
  BCM_COM_PROC_P20/229(V_BCM_COM_RMLG_Inboard_Tire_Press_Cons_Val) -> V_BCM_COM_RMLG_Inboard_Tire_Press_Cons_Val/1
  BCM_COM_PROC_P20/230(V_BCM_COM_RMLG_Outboard_Tire_Press_Cons) -> V_BCM_COM_RMLG_Outboard_Tire_Press_Cons/1
  BCM_COM_PROC_P20/231(V_BCM_COM_RMLG_Outboard_Tire_Press_Cons_Val) -> V_BCM_COM_RMLG_Outboard_Tire_Press_Cons_Val/1
  BCM_COM_PROC_P20/232(V_BCM_COM_A429_SSM_Avionics_Label_005) -> V_BCM_COM_A429_SSM_Avionics_Label_005/1
  BCM_COM_PROC_P20/233(V_BCM_COM_A429_SSM_Avionics_Label_006) -> V_BCM_COM_A429_SSM_Avionics_Label_006/1
  BCM_COM_PROC_P20/234(V_BCM_COM_A429_SSM_Avionics_Label_021) -> V_BCM_COM_A429_SSM_Avionics_Label_021/1
  BCM_COM_PROC_P20/235(V_BCM_COM_A429_SSM_Avionics_Label_022) -> V_BCM_COM_A429_SSM_Avionics_Label_022/1
  BCM_COM_PROC_P20/236(V_BCM_COM_A429_SSM_Avionics_Label_030) -> V_BCM_COM_A429_SSM_Avionics_Label_030/1
  BCM_COM_PROC_P20/237(V_BCM_COM_A429_SSM_Avionics_Label_031) -> V_BCM_COM_A429_SSM_Avionics_Label_031/1
  BCM_COM_PROC_P20/238(V_BCM_COM_A429_SSM_Avionics_Label_032) -> V_BCM_COM_A429_SSM_Avionics_Label_032/1
  BCM_COM_PROC_P20/239(V_BCM_COM_A429_SSM_Avionics_Label_033) -> V_BCM_COM_A429_SSM_Avionics_Label_033/1
  BCM_COM_PROC_P20/240(V_BCM_COM_A429_SSM_Avionics_Label_040) -> V_BCM_COM_A429_SSM_Avionics_Label_040/1
  BCM_COM_PROC_P20/241(V_BCM_COM_A429_SSM_Avionics_Label_041) -> V_BCM_COM_A429_SSM_Avionics_Label_041/1
  BCM_COM_PROC_P20/242(V_BCM_COM_A429_SSM_Avionics_Label_042) -> V_BCM_COM_A429_SSM_Avionics_Label_042/1
  BCM_COM_PROC_P20/243(V_BCM_COM_A429_SSM_Avionics_Label_043) -> V_BCM_COM_A429_SSM_Avionics_Label_043/1
  BCM_COM_PROC_P20/244(V_BCM_COM_A429_SSM_Avionics_Label_050) -> V_BCM_COM_A429_SSM_Avionics_Label_050/1
  BCM_COM_PROC_P20/245(V_BCM_COM_A429_SSM_DFCS_Label_105) -> V_BCM_COM_A429_SSM_DFCS_Label_105/1
  BCM_COM_PROC_P20/246(V_BCM_COM_A429_Wheel_Speed_W12) -> V_BCM_COM_A429_Wheel_Speed_W12/1
  BCM_COM_PROC_P20/247(V_BCM_COM_A429_Wheel_Speed_W34) -> V_BCM_COM_A429_Wheel_Speed_W34/1
  BCM_COM_PROC_P20/248(V_BCM_COM_A429_TACHO_Fail_W12) -> V_BCM_COM_A429_TACHO_Fail_W12/1
  BCM_COM_PROC_P20/249(V_BCM_COM_A429_TACHO_Fail_W34) -> V_BCM_COM_A429_TACHO_Fail_W34/1
  BCM_COM_PROC_P20/250(V_BCM_COM_A429_SSM_Avionics_Label_001) -> V_BCM_COM_A429_SSM_Avionics_Label_001/1
  BCM_COM_PROC_P20/251(V_BCM_COM_A429_SSM_Avionics_Label_002) -> V_BCM_COM_A429_SSM_Avionics_Label_002/1
  BCM_COM_PROC_P20/252(V_BCM_COM_A429_SSM_Avionics_Label_003) -> V_BCM_COM_A429_SSM_Avionics_Label_003/1
  BCM_COM_PROC_P20/253(V_BCM_COM_A429_SSM_Avionics_Label_004) -> V_BCM_COM_A429_SSM_Avionics_Label_004/1
  BCM_COM_PROC_P20/254(V_BCM_COM_A429_SSM_DFCS_Label_101) -> V_BCM_COM_A429_SSM_DFCS_Label_101/1
  BCM_COM_PROC_P20/255(V_BCM_COM_A429_SSM_DFCS_Label_102) -> V_BCM_COM_A429_SSM_DFCS_Label_102/1
  BCM_COM_PROC_P20/256(V_BCM_COM_A429_SSM_DFCS_Label_103) -> V_BCM_COM_A429_SSM_DFCS_Label_103/1
  BCM_COM_PROC_P20/257(V_BCM_COM_A429_SSM_DFCS_Label_104) -> V_BCM_COM_A429_SSM_DFCS_Label_104/1
  BCM_COM_PROC_P20/258(V_BCM_COM_A429_LH_Brake_Temp) -> V_BCM_COM_A429_LH_Brake_Temp/1
  BCM_COM_PROC_P20/259(V_BCM_COM_A429_RH_Brake_Temp) -> V_BCM_COM_A429_RH_Brake_Temp/1
  BCM_COM_PROC_P20/260(V_BCM_COM_A429_LH_Brake_Temp_Sensor_Fail) -> V_BCM_COM_A429_LH_Brake_Temp_Sensor_Fail/1
  BCM_COM_PROC_P20/261(V_BCM_COM_A429_RH_Brake_Temp_Sensor_Fail) -> V_BCM_COM_A429_RH_Brake_Temp_Sensor_Fail/1
  BCM_COM_PROC_P20/262(V_BCM_COM_A429_SSM_Avionics_Label_010) -> V_BCM_COM_A429_SSM_Avionics_Label_010/1
  BCM_COM_PROC_P20/263(V_BCM_COM_A429_SSM_Avionics_Label_011) -> V_BCM_COM_A429_SSM_Avionics_Label_011/1
  BCM_COM_PROC_P20/264(V_BCM_COM_A429_LNLG_Tire_Press) -> V_BCM_COM_A429_LNLG_Tire_Press/1
  BCM_COM_PROC_P20/265(V_BCM_COM_A429_RNLG_Tire_Press) -> V_BCM_COM_A429_RNLG_Tire_Press/1
  BCM_COM_PROC_P20/266(V_BCM_COM_A429_LMLG_Outboard_Tire_Press) -> V_BCM_COM_A429_LMLG_Outboard_Tire_Press/1
  BCM_COM_PROC_P20/267(V_BCM_COM_A429_LMLG_Inboard_Tire_Press) -> V_BCM_COM_A429_LMLG_Inboard_Tire_Press/1
  BCM_COM_PROC_P20/268(V_BCM_COM_A429_RMLG_Inboard_Tire_Press) -> V_BCM_COM_A429_RMLG_Inboard_Tire_Press/1
  BCM_COM_PROC_P20/269(V_BCM_COM_A429_RMLG_Outboard_Tire_Press) -> V_BCM_COM_A429_RMLG_Outboard_Tire_Press/1
  BCM_COM_PROC_P20/270(V_BCM_COM_A429_LNLG_Tire_Press_Sensor_Fail) -> V_BCM_COM_A429_LNLG_Tire_Press_Sensor_Fail/1
  BCM_COM_PROC_P20/271(V_BCM_COM_A429_RNLG_Tire_Press_Sensor_Fail) -> V_BCM_COM_A429_RNLG_Tire_Press_Sensor_Fail/1
  BCM_COM_PROC_P20/272(V_BCM_COM_A429_LMLG_Outboard_Tire_Press_Sensor_Fail) -> V_BCM_COM_A429_LMLG_Outboard_Tire_Press_Sensor_Fail/1
  BCM_COM_PROC_P20/273(V_BCM_COM_A429_LMLG_Inboard_Tire_Press_Sensor_Fail) -> V_BCM_COM_A429_LMLG_Inboard_Tire_Press_Sensor_Fail/1
  BCM_COM_PROC_P20/274(V_BCM_COM_A429_RMLG_Inboard_Tire_Press_Sensor_Fail) -> V_BCM_COM_A429_RMLG_Inboard_Tire_Press_Sensor_Fail/1
  BCM_COM_PROC_P20/275(V_BCM_COM_A429_RMLG_Outboard_Tire_Press_Sensor_Fail) -> V_BCM_COM_A429_RMLG_Outboard_Tire_Press_Sensor_Fail/1
  BCM_COM_PROC_P20/276(V_BCM_COM_A429_TPIS_Fail) -> V_BCM_COM_A429_TPIS_Fail/1
  BCM_COM_PROC_P20/277(V_BCM_COM_A429_SSM_Avionics_Label_012) -> V_BCM_COM_A429_SSM_Avionics_Label_012/1
  BCM_COM_PROC_P20/278(V_BCM_COM_A429_SSM_Avionics_Label_013) -> V_BCM_COM_A429_SSM_Avionics_Label_013/1
  BCM_COM_PROC_P20/279(V_BCM_COM_A429_SSM_Avionics_Label_014) -> V_BCM_COM_A429_SSM_Avionics_Label_014/1
  BCM_COM_PROC_P20/280(V_BCM_COM_A429_SSM_Avionics_Label_015) -> V_BCM_COM_A429_SSM_Avionics_Label_015/1
  BCM_COM_PROC_P20/281(V_BCM_COM_A429_SSM_Avionics_Label_016) -> V_BCM_COM_A429_SSM_Avionics_Label_016/1
  BCM_COM_PROC_P20/282(V_BCM_COM_A429_SSM_Avionics_Label_017) -> V_BCM_COM_A429_SSM_Avionics_Label_017/1
  BCM_COM_PROC_P20/283(V_BCM_COM_A429_Curr_Ord_Before_AS) -> V_BCM_COM_A429_Curr_Ord_Before_AS/1
  BCM_COM_PROC_P20/284(V_BCM_COM_A429_AS_Curr_Order) -> V_BCM_COM_A429_AS_Curr_Order/1
  BCM_COM_PROC_P20/285(V_BCM_COM_A429_SV_Current_Readback) -> V_BCM_COM_A429_SV_Current_Readback/1
  BCM_COM_PROC_P20/286(V_BCM_COM_A429_SV_PT_In_Bar) -> V_BCM_COM_A429_SV_PT_In_Bar/1
  BCM_COM_PROC_P20/287(V_BCM_COM_A429_SV_PT_In_PSI) -> V_BCM_COM_A429_SV_PT_In_PSI/1
  BCM_COM_PROC_P20/288(V_BCM_COM_A429_Antiskid_Activity) -> V_BCM_COM_A429_Antiskid_Activity/1
  BCM_COM_PROC_P20/289(V_BCM_COM_A429_ACCU_PT_Fail) -> V_BCM_COM_A429_ACCU_PT_Fail/1
  BCM_COM_PROC_P20/290(V_BCM_COM_A429_SV_PT_Fail) -> V_BCM_COM_A429_SV_PT_Fail/1
  BCM_COM_PROC_P20/291(V_BCM_COM_A429_SV_Fail) -> V_BCM_COM_A429_SV_Fail/1
  BCM_COM_PROC_P20/292(V_BCM_COM_A429_ACCU_PT) -> V_BCM_COM_A429_ACCU_PT/1
  BCM_COM_PROC_P20/293(V_BCM_COM_A429_SELV_Disc_Sts_Rdbk) -> V_BCM_COM_A429_SELV_Disc_Sts_Rdbk/1
  BCM_COM_PROC_P20/294(V_BCM_COM_A429_SELV_Disc_Sts_Rdbk_Val) -> V_BCM_COM_A429_SELV_Disc_Sts_Rdbk_Val/1
  BCM_COM_PROC_P20/295(V_BCM_COM_A429_SELV_Fail) -> V_BCM_COM_A429_SELV_Fail/1
  BCM_COM_PROC_P20/296(V_BCM_COM_A429_SSM_Avionics_Label_020) -> V_BCM_COM_A429_SSM_Avionics_Label_020/1
  BCM_COM_PROC_P20/297(V_BCM_COM_A429_SSM_Avionics_Label_036) -> V_BCM_COM_A429_SSM_Avionics_Label_036/1
  BCM_COM_PROC_P20/298(V_BCM_COM_A429_SSM_Avionics_Label_037) -> V_BCM_COM_A429_SSM_Avionics_Label_037/1
  BCM_COM_PROC_P20/299(V_BCM_COM_A429_SSM_DFCS_Label_106) -> V_BCM_COM_A429_SSM_DFCS_Label_106/1
  BCM_COM_PROC_P20/300(V_BCM_COM_A429_SSM_DFCS_Label_107) -> V_BCM_COM_A429_SSM_DFCS_Label_107/1
  BCM_COM_PROC_P20/301(V_BCM_COM_A429_SSM_Avionics_Label_034) -> V_BCM_COM_A429_SSM_Avionics_Label_034/1
  BCM_COM_PROC_P20/302(V_BCM_COM_A429_SSM_Avionics_Label_035) -> V_BCM_COM_A429_SSM_Avionics_Label_035/1
  BCM_COM_PROC_P20/303(V_BCM_COM_A429_Park_Brake_ON) -> V_BCM_COM_A429_Park_Brake_ON/1
  BCM_COM_PROC_P20/304(V_BCM_COM_A429_Park_Brake_Fail) -> V_BCM_COM_A429_Park_Brake_Fail/1
  BCM_COM_PROC_P20/305(V_BCM_COM_A429_Norm_FT_In_Progress) -> V_BCM_COM_A429_Norm_FT_In_Progress/1
  BCM_COM_PROC_P20/306(V_BCM_COM_A429_Alt_FT_In_Progress) -> V_BCM_COM_A429_Alt_FT_In_Progress/1
  BCM_COM_PROC_P20/307(V_BCM_COM_A429_Alt_FT_DFCS_Brkg_Req) -> V_BCM_COM_A429_Alt_FT_DFCS_Brkg_Req/1
  BCM_COM_PROC_P20/308(V_BCM_COM_A429_Brk_Residual_Press) -> V_BCM_COM_A429_Brk_Residual_Press/1
  BCM_COM_PROC_P20/309(V_BCM_COM_A429_PLT_Not_Performed) -> V_BCM_COM_A429_PLT_Not_Performed/1
  BCM_COM_PROC_P20/310(V_BCM_COM_A429_Avionics_Comm_Fail_RX) -> V_BCM_COM_A429_Avionics_Comm_Fail_RX/1
  BCM_COM_PROC_P20/311(V_BCM_COM_A429_DFCS_Decel_Law_Inhib) -> V_BCM_COM_A429_DFCS_Decel_Law_Inhib/1
  BCM_COM_PROC_P20/312(V_BCM_COM_A429_LH_Brkg_Cmd_Fdbk) -> V_BCM_COM_A429_LH_Brkg_Cmd_Fdbk/1
  BCM_COM_PROC_P20/313(V_BCM_COM_A429_RH_Brkg_Cmd_Fdbk) -> V_BCM_COM_A429_RH_Brkg_Cmd_Fdbk/1
  BCM_COM_PROC_P20/314(V_BCM_COM_A429_DFCS_LH_Brk_Pdl_Ord_Fail) -> V_BCM_COM_A429_DFCS_LH_Brk_Pdl_Ord_Fail/1
  BCM_COM_PROC_P20/315(V_BCM_COM_A429_DFCS_RH_Brk_Pdl_Ord_Fail) -> V_BCM_COM_A429_DFCS_RH_Brk_Pdl_Ord_Fail/1
  BCM_COM_PROC_P20/316(V_BCM_COM_A429_DFCS_A_Comm_Fail_RX) -> V_BCM_COM_A429_DFCS_A_Comm_Fail_RX/1
  BCM_COM_PROC_P20/317(V_BCM_COM_A429_DFCS_B_Comm_Fail_RX) -> V_BCM_COM_A429_DFCS_B_Comm_Fail_RX/1
  BCM_COM_PROC_P20/318(V_BCM_COM_A429_DFCS_A_Capsule_Fail) -> V_BCM_COM_A429_DFCS_A_Capsule_Fail/1
  BCM_COM_PROC_P20/319(V_BCM_COM_A429_DFCS_B_Capsule_Fail) -> V_BCM_COM_A429_DFCS_B_Capsule_Fail/1
  BCM_COM_PROC_P20/320(V_BCM_COM_A429_Pinprog_1) -> V_BCM_COM_A429_Pinprog_1/1
  BCM_COM_PROC_P20/321(V_BCM_COM_A429_Pinprog_2) -> V_BCM_COM_A429_Pinprog_2/1
  BCM_COM_PROC_P20/322(V_BCM_COM_A429_Pinprog_3) -> V_BCM_COM_A429_Pinprog_3/1
  BCM_COM_PROC_P20/323(V_BCM_COM_A429_Pinprog_4) -> V_BCM_COM_A429_Pinprog_4/1
  BCM_COM_PROC_P20/324(V_BCM_COM_A429_Pinprog_5) -> V_BCM_COM_A429_Pinprog_5/1
  BCM_COM_PROC_P20/325(V_BCM_COM_A429_PP_Channel_ID) -> V_BCM_COM_A429_PP_Channel_ID/1
  BCM_COM_PROC_P20/326(V_BCM_COM_A429_DBCU_Dispatch_Conf) -> V_BCM_COM_A429_DBCU_Dispatch_Conf/1
  BCM_COM_PROC_P20/327(V_BCM_COM_A429_Maint_Mode_Active) -> V_BCM_COM_A429_Maint_Mode_Active/1
  BCM_COM_PROC_P20/328(V_BCM_COM_A429_Maint_Mode_Req_GND) -> V_BCM_COM_A429_Maint_Mode_Req_GND/1
  BCM_COM_PROC_P20/329(V_BCM_COM_A429_Maint_Mode_Req_28V) -> V_BCM_COM_A429_Maint_Mode_Req_28V/1
  BCM_COM_PROC_P20/330(V_BCM_COM_A429_Pinprog_Fail) -> V_BCM_COM_A429_Pinprog_Fail/1
  BCM_COM_PROC_P20/331(V_BCM_COM_A429_Norm_Brake_Fail) -> V_BCM_COM_A429_Norm_Brake_Fail/1
  BCM_COM_PROC_P20/332(V_BCM_COM_A429_BCM_Passivated) -> V_BCM_COM_A429_BCM_Passivated/1
  BCM_COM_PROC_P20/333(V_BCM_COM_A429_BCM_Fail) -> V_BCM_COM_A429_BCM_Fail/1
  BCM_COM_PROC_P20/334(V_BCM_COM_A429_DBCU_Fail) -> V_BCM_COM_A429_DBCU_Fail/1
  BCM_COM_PROC_P20/335(V_BCM_COM_A429_Alternate_Fail) -> V_BCM_COM_A429_Alternate_Fail/1
  BCM_COM_PROC_P20/336(V_BCM_COM_A429_DBCU_LH_Brk_Cmd_Fdbk) -> V_BCM_COM_A429_DBCU_LH_Brk_Cmd_Fdbk/1
  BCM_COM_PROC_P20/337(V_BCM_COM_A429_DBCU_RH_Brk_Cmd_Fdbk) -> V_BCM_COM_A429_DBCU_RH_Brk_Cmd_Fdbk/1
  BCM_COM_PROC_P20/338(V_BCM_COM_A429_DBCU_Inhib_Opp_Side) -> V_BCM_COM_A429_DBCU_Inhib_Opp_Side/1
  BCM_COM_PROC_P20/339(V_BCM_COM_A429_DBCU_Alt_Mode) -> V_BCM_COM_A429_DBCU_Alt_Mode/1
  BCM_COM_PROC_P20/340(V_BCM_COM_A429_SSM_DFCS_Label_100) -> V_BCM_COM_A429_SSM_DFCS_Label_100/1
  BCM_COM_PROC_P20/341(V_BCM_COM_A429_Global_Wheel_Spd) -> V_BCM_COM_A429_Global_Wheel_Spd/1
  BCM_COM_PROC_P20/342(V_BCM_COM_ETH_HYD_A_PRESS) -> V_BCM_COM_ETH_HYD_A_PRESS/1
  BCM_COM_PROC_P20/343(V_BCM_COM_ETH_HYD_B_PRESS) -> V_BCM_COM_ETH_HYD_B_PRESS/1
  BCM_COM_PROC_P20/344(V_BCM_COM_ETH_ENG1_RUNNING) -> V_BCM_COM_ETH_ENG1_RUNNING/1
  BCM_COM_PROC_P20/345(V_BCM_COM_ETH_ENG2_RUNNING) -> V_BCM_COM_ETH_ENG2_RUNNING/1
  BCM_COM_PROC_P20/346(V_BCM_COM_ETH_LMLG_Dnlk) -> V_BCM_COM_ETH_LMLG_Dnlk/1
  BCM_COM_PROC_P20/347(V_BCM_COM_ETH_RMLG_Dnlk) -> V_BCM_COM_ETH_RMLG_Dnlk/1
  BCM_COM_PROC_P20/348(V_BCM_COM_ETH_Lever_Up) -> V_BCM_COM_ETH_Lever_Up/1
  BCM_COM_PROC_P20/349(V_BCM_COM_ETH_BCP_BCM_ALT_SW_ON_CMD) -> V_BCM_COM_ETH_BCP_BCM_ALT_SW_ON_CMD/1
  BCM_COM_PROC_P20/350(V_BCM_COM_ETH_MP_MAINT_MODE_CMD_GND) -> V_BCM_COM_ETH_MP_MAINT_MODE_CMD_GND/1
  BCM_COM_PROC_P20/351(V_BCM_COM_ETH_MP_MAINT_MODE_CMD_28V) -> V_BCM_COM_ETH_MP_MAINT_MODE_CMD_28V/1
  BCM_COM_PROC_P20/352(V_BCM_COM_ETH_MP_BCMA_ALT_DISP_SW) -> V_BCM_COM_ETH_MP_BCMA_ALT_DISP_SW/1
  BCM_COM_PROC_P20/353(V_BCM_COM_ETH_PBSELV_ON_POS) -> V_BCM_COM_ETH_PBSELV_ON_POS/1
  BCM_COM_PROC_P20/354(V_BCM_COM_ETH_DBCU_BRK_ORDER_FAIL) -> V_BCM_COM_ETH_DBCU_BRK_ORDER_FAIL/1
  BCM_COM_PROC_P20/355(V_BCM_COM_ETH_DISPATCH_SW_ON) -> V_BCM_COM_ETH_DISPATCH_SW_ON/1
  BCM_COM_PROC_P20/356(V_BCM_COM_ETH_LH_DBCU_BRK_CMD_FDBK) -> V_BCM_COM_ETH_LH_DBCU_BRK_CMD_FDBK/1
  BCM_COM_PROC_P20/357(V_BCM_COM_ETH_RH_DBCU_BRK_CMD_FDBK) -> V_BCM_COM_ETH_RH_DBCU_BRK_CMD_FDBK/1
  BCM_COM_PROC_P20/358(V_BCM_COM_ETH_DBCU_FAILED) -> V_BCM_COM_ETH_DBCU_FAILED/1
  BCM_COM_PROC_P20/359(V_BCM_COM_ETH_ALT_MODE) -> V_BCM_COM_ETH_ALT_MODE/1
  BCM_COM_PROC_P20/360(V_BCM_COM_ETH_Opp_BCM_DBCU_INHIB) -> V_BCM_COM_ETH_Opp_BCM_DBCU_INHIB/1
  BCM_COM_PROC_P20/361(V_BCM_COM_ETH_LH_SV_Current_Order) -> V_BCM_COM_ETH_LH_SV_Current_Order/1
  BCM_COM_PROC_P20/362(V_BCM_COM_ETH_RH_SV_Current_Order) -> V_BCM_COM_ETH_RH_SV_Current_Order/1
  BCM_COM_PROC_P20/363(V_BCM_COM_ETH_SELV_High_Side_Cmd_Order) -> V_BCM_COM_ETH_SELV_High_Side_Cmd_Order/1
  BCM_COM_PROC_P20/364(V_BCM_COM_ETH_DBCU_Inhib_Order) -> V_BCM_COM_ETH_DBCU_Inhib_Order/1
  BCM_COM_PROC_P20/365(V_BCM_COM_ETH_FB_BCM_FAIL) -> V_BCM_COM_ETH_FB_BCM_FAIL/1
  BCM_COM_PROC_P20/366(V_BCM_COM_ETH_FB_DFCS_A_RX) -> V_BCM_COM_ETH_FB_DFCS_A_RX/1
  BCM_COM_PROC_P20/367(V_BCM_COM_ETH_FB_DFCS_B_RX) -> V_BCM_COM_ETH_FB_DFCS_B_RX/1
  BCM_COM_PROC_P20/368(V_BCM_COM_ETH_FB_MAINT_MODE_DIS) -> V_BCM_COM_ETH_FB_MAINT_MODE_DIS/1
  BCM_COM_PROC_P20/369(V_BCM_COM_ETH_FB_PARK_BRK_STATUS_DIS) -> V_BCM_COM_ETH_FB_PARK_BRK_STATUS_DIS/1
  BCM_COM_PROC_P20/370(V_BCM_COM_ETH_FB_BCM_DBCU_MODE_DIS) -> V_BCM_COM_ETH_FB_BCM_DBCU_MODE_DIS/1
  BCM_COM_PROC_P20/371(V_BCM_COM_ETH_FB_DBCU_SIMULT_ACT) -> V_BCM_COM_ETH_FB_DBCU_SIMULT_ACT/1
  BCM_COM_PROC_P20/372(V_BCM_COM_ETH_FB_DBCU_FAIL) -> V_BCM_COM_ETH_FB_DBCU_FAIL/1
  BCM_COM_PROC_P20/373(V_BCM_COM_ETH_FB_DBCU_BRK_ORDER_FAIL) -> V_BCM_COM_ETH_FB_DBCU_BRK_ORDER_FAIL/1
  BCM_COM_PROC_P20/374(V_BCM_COM_ETH_FB_INHIB_FAIL) -> V_BCM_COM_ETH_FB_INHIB_FAIL/1
  BCM_COM_PROC_P20/375(V_BCM_COM_ETH_FB_HYD_A_LOW_PRESS) -> V_BCM_COM_ETH_FB_HYD_A_LOW_PRESS/1
  BCM_COM_PROC_P20/376(V_BCM_COM_ETH_FB_HYD_B_LOW_PRESS) -> V_BCM_COM_ETH_FB_HYD_B_LOW_PRESS/1
  BCM_COM_PROC_P20/377(V_BCM_COM_ETH_FB_ACCU_LOW_PRESS) -> V_BCM_COM_ETH_FB_ACCU_LOW_PRESS/1
  BCM_COM_PROC_P20/378(V_BCM_COM_ETH_FB_ACCU_PT_FAIL) -> V_BCM_COM_ETH_FB_ACCU_PT_FAIL/1
  BCM_COM_PROC_P20/379(V_BCM_COM_ETH_FB_BSELV_CMD_FAIL) -> V_BCM_COM_ETH_FB_BSELV_CMD_FAIL/1
  BCM_COM_PROC_P20/380(V_BCM_COM_ETH_FB_BSELV_JCL) -> V_BCM_COM_ETH_FB_BSELV_JCL/1
  BCM_COM_PROC_P20/381(V_BCM_COM_ETH_FB_BSELV_JOP) -> V_BCM_COM_ETH_FB_BSELV_JOP/1
  BCM_COM_PROC_P20/382(V_BCM_COM_ETH_FB_LH_SV_PT_FAIL) -> V_BCM_COM_ETH_FB_LH_SV_PT_FAIL/1
  BCM_COM_PROC_P20/383(V_BCM_COM_ETH_FB_LH_SV_CMD_FAIL) -> V_BCM_COM_ETH_FB_LH_SV_CMD_FAIL/1
  BCM_COM_PROC_P20/384(V_BCM_COM_ETH_FB_LH_SV_JCL) -> V_BCM_COM_ETH_FB_LH_SV_JCL/1
  BCM_COM_PROC_P20/385(V_BCM_COM_ETH_FB_LH_SV_JOP) -> V_BCM_COM_ETH_FB_LH_SV_JOP/1
  BCM_COM_PROC_P20/386(V_BCM_COM_ETH_FB_RH_SV_PT_FAIL) -> V_BCM_COM_ETH_FB_RH_SV_PT_FAIL/1
  BCM_COM_PROC_P20/387(V_BCM_COM_ETH_FB_RH_SV_CMD_FAIL) -> V_BCM_COM_ETH_FB_RH_SV_CMD_FAIL/1
  BCM_COM_PROC_P20/388(V_BCM_COM_ETH_FB_RH_SV_JCL) -> V_BCM_COM_ETH_FB_RH_SV_JCL/1
  BCM_COM_PROC_P20/389(V_BCM_COM_ETH_FB_RH_SV_JOP) -> V_BCM_COM_ETH_FB_RH_SV_JOP/1
  BCM_COM_PROC_P20/390(V_BCM_COM_ETH_AC_State) -> V_BCM_COM_ETH_AC_State/1
  BCM_COM_PROC_P20/391(V_BCM_COM_ETH_AC_Flight_Phase) -> V_BCM_COM_ETH_AC_Flight_Phase/1
  BCM_COM_PROC_P20/392(V_BCM_COM_ETH_Braking_Mode) -> V_BCM_COM_ETH_Braking_Mode/1
  BCM_COM_PROC_P20/393(V_BCM_COM_ETH_Braking_Norm_FT_Seq) -> V_BCM_COM_ETH_Braking_Norm_FT_Seq/1
  BCM_COM_PROC_P20/394(V_BCM_COM_ETH_Braking_Alt_FT_Seq) -> V_BCM_COM_ETH_Braking_Alt_FT_Seq/1
  BCM_COM_PROC_P20/395(V_BCM_COM_ETH_FB_LG_LEVER_FAIL) -> V_BCM_COM_ETH_FB_LG_LEVER_FAIL/1
  BCM_COM_PROC_P20/396(V_BCM_COM_ETH_FB_LMLG_DWNLOCK_FAIL) -> V_BCM_COM_ETH_FB_LMLG_DWNLOCK_FAIL/1
  BCM_COM_PROC_P20/397(V_BCM_COM_ETH_FB_RMLG_DWNLOCK_FAIL) -> V_BCM_COM_ETH_FB_RMLG_DWNLOCK_FAIL/1
  BCM_COM_PROC_P20/398(V_BCM_COM_ETH_TARGET_HW_ID) -> V_BCM_COM_ETH_TARGET_HW_ID/1
  BCM_COM_PROC_P20/399(V_BCM_COM_ETH_Invalid_Config) -> V_BCM_COM_ETH_Invalid_Config/1
  BCM_COM_PROC_P20/400(V_BCM_COM_ETH_FB_LH_OUT_TACHO_FAIL) -> V_BCM_COM_ETH_FB_LH_OUT_TACHO_FAIL/1
  BCM_COM_PROC_P20/401(V_BCM_COM_ETH_FB_LH_IN_TACHO_FAIL) -> V_BCM_COM_ETH_FB_LH_IN_TACHO_FAIL/1
  BCM_COM_PROC_P20/402(V_BCM_COM_ETH_FB_RH_IN_TACHO_FAIL) -> V_BCM_COM_ETH_FB_RH_IN_TACHO_FAIL/1
  BCM_COM_PROC_P20/403(V_BCM_COM_ETH_FB_RH_OUT_TACHO_FAIL) -> V_BCM_COM_ETH_FB_RH_OUT_TACHO_FAIL/1
  BCM_COM_PROC_P20/404(V_BCM_COM_ETH_TT_in_progress_id) -> V_BCM_COM_ETH_TT_in_progress_id/1
  BCM_COM_PROC_P20/405(V_BCM_COM_ETH_TT_rejection_cause) -> V_BCM_COM_ETH_TT_rejection_cause/1
  BCM_COM_PROC_P20/406(V_BCM_COM_ETH_TT_rejected) -> V_BCM_COM_ETH_TT_rejected/1
  BCM_COM_PROC_P20/407(V_BCM_COM_ETH_TT_completed) -> V_BCM_COM_ETH_TT_completed/1
  BCM_COM_PROC_P20/408(V_BCM_COM_ETH_TT_result_significant) -> V_BCM_COM_ETH_TT_result_significant/1
  BCM_COM_PROC_P20/409(V_BCM_COM_BCM_DBCU_INHIBITION_Conf) -> V_BCM_COM_BCM_DBCU_INHIBITION_Conf/1
  BCM_COM_PROC_P20/410(V_BCM_COM_Target_DCL) -> V_BCM_COM_Target_DCL/1
  BCM_COM_PROC_P20/411(V_BCM_COM_Decel_Ctrl_Loop_Act_Cond) -> V_BCM_COM_Decel_Ctrl_Loop_Act_Cond/1
